simulink model "MGmono_rtiFPGASeparationFile"  (R2018b)
settings: Solver=FixedStepAuto  StartTime=0.0  StopTime=Inf  FixedStep=N*T  RelTol=1e-3
PostLoadFcn:
  | , if any(exist('dsrtsu_mdlpostloadfcn', 'file') ~= 0), dsrtsu_mdlpostloadfcn('Execute', bdroot); end,
InitFcn:
  | , if any(exist('dsmpb_private', 'file') ~= 0), dsmpb_private('dsmpb_mdlclblib', 'Init', bdroot); end,
values from neighbouring files (symbols this model uses):
  amp = 1    [param.m]
  fixedgain_i = 10*1000/(3*100)    (= 33.3333333333)    [param.m]
  fixedgain_vc1 = 10*10000/(3*100*2.5)    (= 133.333333333)    [param.m]
  fixedgain_vc2 = 10*10000/(3*100*2.5)    (= 133.333333333)    [param.m]
  fixedgain_vc3 = 10*22000/(3*100*2.5)    (= 293.333333333)    [param.m]
  fixedgain_vc4 = 10*22000/(3*100*2.5)    (= 293.333333333)    [param.m]
  fixedgain_vc5 = 10*22000/(3*100*2.5)    (= 293.333333333)    [param.m]
  freq = 50    [param.m]
  gain_iL1 = 1    [param.m]
  gain_iL2 = 1    [param.m]
  gain_iL3 = 1    [param.m]
  gain_iL4 = 1    [param.m]
  gain_vc1 = 1    [param.m]
  gain_vc2 = 1    [param.m]
  gain_vc3 = 1    [param.m]
  gain_vc4 = 1    [param.m]
  gain_vc5 = 1    [param.m]
  Ii = 10    [param.m]
  Ipv = 0.01    [param.m]
  Iv = 0.1    [param.m]
  Ki = 1e-7    (= 1e-07)    [param.m]
  Kp = 0.5    [param.m]
  maxd = N-1    (= 9)    [param.m]
  mind = 1    [param.m]
  N = 10    [param.m]
  offset_iL1 = 0.2    [param.m]
  offset_iL2 = 0.2    [param.m]
  offset_iL3 = -2e-3    (= -0.002)    [param.m]
  offset_iL4 = -2e-3    (= -0.002)    [param.m]
  offset_vc1 = -0.21    [param.m]
  offset_vc2 = -0.17    [param.m]
  offset_vc3 = 0.2    [param.m]
  offset_vc4 = -0.05    [param.m]
  offset_vc5 = -0.01    [param.m]
  Pi = 0.3    [param.m]
  Ppv = 0.05    [param.m]
  Pv = 0.01    [param.m]
  T = 6e-6    (= 6e-06)    [param.m]
  Tf = 1/1000    (= 0.001)    [param.m]
  Tfdc = 1/20    (= 0.05)    [param.m]
  v_dc_ref = 80    [param.m]
undefined symbols (not defined in the file or in its folder): DiscIntNeverNeededParam
libraries: xbsIndex_r4 x155, rti1202lib_adc_class1 x9, rtiproclib x7, simulink x6, rtifpgainterfacelib x1
(part 3 of 5)

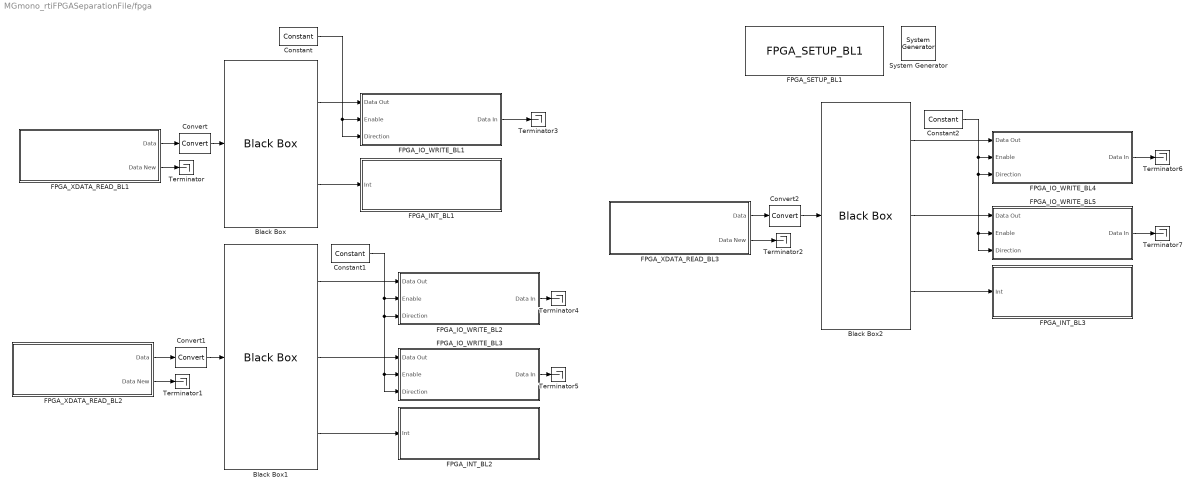
== system MGmono_rtiFPGASeparationFile/fpga ==
  " System Generator" : xbsIndex_r4/ System Generator  Tag=genX  xilinxfamily=kintex7  part=xc7k325t  speed=-3  package=fbg676  synthesis_tool=Vivado  clock_wrapper=Clock Enables  directory=./netlist  proj_type=Vivado  Synth_file=Vivado Synthesis Defaults  Impl_file=Vivado Implementation Defaults  testbench=off  simulink_period=1e-08  sysclk_period=10  dcm_input_clock_period=10  incr_netlist=off  trim_vbits=Everywhere in SubSystem  dbl_ovrd=According to Block Masks  core_generation=According to Block Masks  run_coregen=off  deprecated_control=off  eval_field=0  block_type=sysgen
  Black Box : xbsIndex_r4/Black Box  init_code=boost_config  sim_method=ISE Simulator  verbose=off  block_type=blackbox2
  Black Box1 : xbsIndex_r4/Black Box  init_code=halfbridge_config  sim_method=ISE Simulator  verbose=off  block_type=blackbox2
  Black Box2 : xbsIndex_r4/Black Box  init_code=hb_inv_config  sim_method=ISE Simulator  verbose=off  block_type=blackbox2
  Constant : xbsIndex_r4/Constant  const=1.0  gui_display_data_type=Fixed-point  arith_type=Signed (2's comp)  n_bits=16  bin_pt=14  preci_type=Single  exp_width=8  frac_width=24  explicit_period=off  period=1  equ=P=C  opselect=C  inp2=PCIN>>17  opr=+  inp1=P  carry=CIN  dbl_ovrd=off  block_type=constant
  Constant1 : xbsIndex_r4/Constant  const=1.0  gui_display_data_type=Fixed-point  arith_type=Signed (2's comp)  n_bits=16  bin_pt=14  preci_type=Single  exp_width=8  frac_width=24  explicit_period=off  period=1  equ=P=C  opselect=C  inp2=PCIN>>17  opr=+  inp1=P  carry=CIN  dbl_ovrd=off  block_type=constant
  Constant2 : xbsIndex_r4/Constant  const=1.0  gui_display_data_type=Fixed-point  arith_type=Signed (2's comp)  n_bits=16  bin_pt=14  preci_type=Single  exp_width=8  frac_width=24  explicit_period=off  period=1  equ=P=C  opselect=C  inp2=PCIN>>17  opr=+  inp1=P  carry=CIN  dbl_ovrd=off  block_type=constant
  Convert : xbsIndex_r4/Convert  gui_display_data_type=Fixed-point  arith_type=Unsigned  n_bits=10  bin_pt=0  float_type=Single  exp_bits=8  fraction_bits=24  quantization=Truncate  overflow=Wrap  en=off  latency=1  pipeline=off  dbl_ovrd=off  block_type=convert
  Convert1 : xbsIndex_r4/Convert  gui_display_data_type=Fixed-point  arith_type=Unsigned  n_bits=10  bin_pt=0  float_type=Single  exp_bits=8  fraction_bits=24  quantization=Truncate  overflow=Wrap  en=off  latency=1  pipeline=off  dbl_ovrd=off  block_type=convert
  Convert2 : xbsIndex_r4/Convert  gui_display_data_type=Fixed-point  arith_type=Unsigned  n_bits=10  bin_pt=0  float_type=Single  exp_bits=8  fraction_bits=24  quantization=Truncate  overflow=Wrap  en=off  latency=1  pipeline=off  dbl_ovrd=off  block_type=convert
  FPGA_INT_BL1 : Subsystem  LoadFcn=try, rti_fpga_blk_loadfcn(gcbh); catch,errordlg({lasterr, '','Please check your RTI installation.'},['Error: ' upper(bdroot)], 'replace'); end  InitFcn=try, rti_fpga_blk_initfcn(gcbh); catch,errordlg({lasterr, '','Please check your RTI installation.'},['Error: ' upper(bdroot)], 'replace'); end  StartFcn=try, rti_fpga_blk_startfcn(gcbh); catch,errordlg({lasterr, '','Please check your RTI installation.'},['Error: ' upper(bdroot)], 'replace'); end  mask(RTI){DSProperties=struct('RTI',struct('Version',uint32(4),'BlockType',struct('isSLSource',uint8(0),'isSLSink',uint8(0),'isHWSource',uint8(0),'isHWSink',uint8(0),'isSetup',uint8(1),'isInline',uint8(1),'isNonInline',uint8(0),'isInterrupt',uint8(0),'isChannelwise',uint8(0)),'IOBoardType','DSFPGA','UnitType','','Identifier','INT','DialogType','ML','BlockSet','FPGA','SlaveProcessor','')), RTIBlockInterface=struct('InputPortsActive',1,'InputPortsWidth',int32(1),'InputPortsDataType',{{'SS_DOUBLE'}},'InputPortsName',{{'Int'}},'InitLevel',3,'DialogFcn','rtifpgaintgui','BlockDisplay',{{'Interrupt','auto'}},'IconTransparency','on','BlockName',struct('Token',{{'FPGA_INT_BL1'}})), RTIBlockParameters=struct('BoardNo',{{1,'OFF',[1 16]}},'Name',{{['Interrupt 1'],'OFF',[]}},'CustomName',{{['int_pv '],'OFF',[]}},'AccessTyp',{{'Interrupt','OFF',[]}},'ChannelNo',{{'1','OFF',[]}},'FrmIni',{{'fpga_framework_ini_DS1302_XC7K325T_FLEXIBLEIO','OFF',[]}},'DynFcn',{{struct('GUIPar',struct('Name',{{['Enable simulation port']},{'Used'}},'GUIType',{{'checkbox'},{'none'}},'Range',{{'0','1'},{'0','1'}},'Init',{{'0'},{'1','0'}},'Group',{{''},{''}},'Generic',{{''},{'usr_int_00_used'}},'Application',{{'ApplicationIn(1).Show'},{''}},'Framework',{{''},{''}},'Callback',{{''},{''}}),'Exl',{{''}},'HlpFile',{{'rtifpga','INT_OUT_DS1302'}},'Hlp',{{['Click below for further details on this I/O function.']}},'Gen',struct('name',{'','usr_int_00_used'},'value',{'','1'},'unusedinit',{'','0'},'tag',{'',''},'filename',{'',''}),'Frm',struct('FrameworkOut',struct('Name',{{'usr_interrupt_00'}},'BitWidth',{{'1'}},'BinaryPoint',{{'0'}},'Format',{{'unsigned'}}),'FrameworkIn',struct('Name',{},'BitWidth',{},'BinaryPoint',{},'Format',{})),'App',struct('ApplicationOut',struct('Name',{{'Int'}},'Show',{{true}}),'ApplicationIn',struct('Name',{{'Sim_Int'}},'Show',{{0}})),'Con',{{'FrameworkOut(1)','ApplicationOut(1)'}},'OffCon',{{'data_i','FrameworkOut(1)','data_o','ApplicationIn(1)'}},'OffModel',{{'phs_interrupt'}}),'OFF',[]}},'FPGAFrameworkId',{{'8','OFF',[]}},'CorrBlock',{{struct('Data','','DataTag',''),'OFF',[]}}), RTISFcnParameters=struct('BoardNo','double'), RTIBlockParaDefault=struct('BoardNo',1,'Name',[' '],'CustomName',[' '],'AccessTyp',['<not selected>'],'ChannelNo',['<not selected>'],'FrmIni',[' '],'DynFcn',struct('GUIPar','','Hlp','','HlpFile','','Frm','','Gen','','Exl','','App','','Con',''),'FPGAFrameworkId',[' '],'CorrBlock',struct('Data','','DataTag',''))}
      mask init:
      | % blkh = gcbh;
      | % [sfi, sfp, sfpt] = rti_fpga_blockinitial(blkh,'UPDATEPARAMETER');
      | % rti_fpga_blockinitial(blkh,'UPDATEBLOCKGUI');
      settings: CopyFcn=try, rti_fpga_blk_copyfcn(gcbh); catch,errordlg({lasterr, '','Please check your RTI installation.'},['Error: ' upper(bdroot)], 'replace'); end  DeleteFcn=try, rti_fpga_blk_deletefcn(gcbh); catch,errordlg({lasterr, '','Please check your RTI installation.'},['Error: ' upper(bdroot)], 'replace'); end  ModelCloseFcn=try, rti_fpga_blk_modelclosefcn(gcbh); catch,errordlg({lasterr, '','Please check your RTI installation.'},['Error: ' upper(bdroot)], 'replace'); end  PreSaveFcn=try, rti_fpga_blk_presavefcn(gcbh); catch,errordlg({lasterr, '','Please check your RTI installation.'},['Error: ' upper(bdroot)], 'replace'); end  NameChangeFcn=try, rti_fpga_blk_namechangefcn(gcbh); catch,errordlg({lasterr, '','Please check your RTI installation.'},['Error: ' upper(bdroot)], 'replace'); end  OpenFcn=try, rti_fpga_blk_openfcn(gcbh); catch,errordlg({lasterr, '','Please check your RTI installation.'},['Error: ' upper(bdroot)], 'replace'); end  CloseFcn=try, rti_fpga_blk_closefcn(gcbh); catch,errordlg({lasterr, '','Please check your RTI installation.'},['Error: ' upper(bdroot)], 'replace'); end  ParentCloseFcn=try, rti_fpga_blk_parentclosefcn(gcbh); catch,errordlg({lasterr, '','Please check your RTI installation.'},['Error: ' upper(bdroot)], 'replace'); end
      mask Help: eval( ['lasterror(''reset''); rtifpgaguilib(''RTIMaskHelp'', gcbh);', 'disp(lasterr);']);
      mask Display: text(0.5,0.575,'Interrupt 1','HorizontalAlignment','center');text(0.5,0.425,'int_pv ','HorizontalAlignment','center');
  FPGA_INT_BL2 : Subsystem  LoadFcn=try, rti_fpga_blk_loadfcn(gcbh); catch,errordlg({lasterr, '','Please check your RTI installation.'},['Error: ' upper(bdroot)], 'replace'); end  InitFcn=try, rti_fpga_blk_initfcn(gcbh); catch,errordlg({lasterr, '','Please check your RTI installation.'},['Error: ' upper(bdroot)], 'replace'); end  StartFcn=try, rti_fpga_blk_startfcn(gcbh); catch,errordlg({lasterr, '','Please check your RTI installation.'},['Error: ' upper(bdroot)], 'replace'); end  mask(RTI){DSProperties=struct('RTI',struct('Version',uint32(4),'BlockType',struct('isSLSource',uint8(0),'isSLSink',uint8(0),'isHWSource',uint8(0),'isHWSink',uint8(0),'isSetup',uint8(1),'isInline',uint8(1),'isNonInline',uint8(0),'isInterrupt',uint8(0),'isChannelwise',uint8(0)),'IOBoardType','DSFPGA','UnitType','','Identifier','INT','DialogType','ML','BlockSet','FPGA','SlaveProcessor','')), RTIBlockInterface=struct('InputPortsActive',1,'InputPortsWidth',int32(1),'InputPortsDataType',{{'SS_DOUBLE'}},'InputPortsName',{{'Int'}},'InitLevel',3,'DialogFcn','rtifpgaintgui','BlockDisplay',{{'Interrupt','auto'}},'IconTransparency','on','BlockName',struct('Token',{{'FPGA_INT_BL1'}})), RTIBlockParameters=struct('BoardNo',{{1,'OFF',[1 16]}},'Name',{{['Interrupt 2'],'OFF',[]}},'CustomName',{{'int_bat','OFF',[]}},'AccessTyp',{{'Interrupt','OFF',[]}},'ChannelNo',{{'2','OFF',[]}},'FrmIni',{{'fpga_framework_ini_DS1302_XC7K325T_FLEXIBLEIO','OFF',[]}},'DynFcn',{{struct('GUIPar',struct('Name',{{['Enable simulation port']},{'Used'}},'GUIType',{{'checkbox'},{'none'}},'Range',{{'0','1'},{'0','1'}},'Init',{{'0'},{'1','0'}},'Group',{{''},{''}},'Generic',{{''},{'usr_int_01_used'}},'Application',{{'ApplicationIn(1).Show'},{''}},'Framework',{{''},{''}},'Callback',{{''},{''}}),'Exl',{{''}},'HlpFile',{{'rtifpga','INT_OUT_DS1302'}},'Hlp',{{['Click below for further details on this I/O function.']}},'Gen',struct('name',{'','usr_int_01_used'},'value',{'','1'},'unusedinit',{'','0'},'tag',{'',''},'filename',{'',''}),'Frm',struct('FrameworkOut',struct('Name',{{'usr_interrupt_01'}},'BitWidth',{{'1'}},'BinaryPoint',{{'0'}},'Format',{{'unsigned'}}),'FrameworkIn',struct('Name',{},'BitWidth',{},'BinaryPoint',{},'Format',{})),'App',struct('ApplicationOut',struct('Name',{{'Int'}},'Show',{{true}}),'ApplicationIn',struct('Name',{{'Sim_Int'}},'Show',{{0}})),'Con',{{'FrameworkOut(1)','ApplicationOut(1)'}},'OffCon',{{'data_i','FrameworkOut(1)','data_o','ApplicationIn(1)'}},'OffModel',{{'phs_interrupt'}}),'OFF',[]}},'FPGAFrameworkId',{{'8','OFF',[]}},'CorrBlock',{{struct('Data','','DataTag',''),'OFF',[]}}), RTISFcnParameters=struct('BoardNo','double'), RTIBlockParaDefault=struct('BoardNo',1,'Name',[' '],'CustomName',[' '],'AccessTyp',['<not selected>'],'ChannelNo',['<not selected>'],'FrmIni',[' '],'DynFcn',struct('GUIPar','','Hlp','','HlpFile','','Frm','','Gen','','Exl','','App','','Con',''),'FPGAFrameworkId',[' '],'CorrBlock',struct('Data','','DataTag',''))}
      mask init:
      | % blkh = gcbh;
      | % [sfi, sfp, sfpt] = rti_fpga_blockinitial(blkh,'UPDATEPARAMETER');
      | % rti_fpga_blockinitial(blkh,'UPDATEBLOCKGUI');
      settings: CopyFcn=try, rti_fpga_blk_copyfcn(gcbh); catch,errordlg({lasterr, '','Please check your RTI installation.'},['Error: ' upper(bdroot)], 'replace'); end  DeleteFcn=try, rti_fpga_blk_deletefcn(gcbh); catch,errordlg({lasterr, '','Please check your RTI installation.'},['Error: ' upper(bdroot)], 'replace'); end  ModelCloseFcn=try, rti_fpga_blk_modelclosefcn(gcbh); catch,errordlg({lasterr, '','Please check your RTI installation.'},['Error: ' upper(bdroot)], 'replace'); end  PreSaveFcn=try, rti_fpga_blk_presavefcn(gcbh); catch,errordlg({lasterr, '','Please check your RTI installation.'},['Error: ' upper(bdroot)], 'replace'); end  NameChangeFcn=try, rti_fpga_blk_namechangefcn(gcbh); catch,errordlg({lasterr, '','Please check your RTI installation.'},['Error: ' upper(bdroot)], 'replace'); end  OpenFcn=try, rti_fpga_blk_openfcn(gcbh); catch,errordlg({lasterr, '','Please check your RTI installation.'},['Error: ' upper(bdroot)], 'replace'); end  CloseFcn=try, rti_fpga_blk_closefcn(gcbh); catch,errordlg({lasterr, '','Please check your RTI installation.'},['Error: ' upper(bdroot)], 'replace'); end  ParentCloseFcn=try, rti_fpga_blk_parentclosefcn(gcbh); catch,errordlg({lasterr, '','Please check your RTI installation.'},['Error: ' upper(bdroot)], 'replace'); end
      mask Help: eval( ['lasterror(''reset''); rtifpgaguilib(''RTIMaskHelp'', gcbh);', 'disp(lasterr);']);
      mask Display: text(0.5,0.575,'Interrupt 2','HorizontalAlignment','center');text(0.5,0.425,'int_bat','HorizontalAlignment','center');
  FPGA_INT_BL3 : Subsystem  LoadFcn=try, rti_fpga_blk_loadfcn(gcbh); catch,errordlg({lasterr, '','Please check your RTI installation.'},['Error: ' upper(bdroot)], 'replace'); end  InitFcn=try, rti_fpga_blk_initfcn(gcbh); catch,errordlg({lasterr, '','Please check your RTI installation.'},['Error: ' upper(bdroot)], 'replace'); end  StartFcn=try, rti_fpga_blk_startfcn(gcbh); catch,errordlg({lasterr, '','Please check your RTI installation.'},['Error: ' upper(bdroot)], 'replace'); end  mask(RTI){DSProperties=struct('RTI',struct('Version',uint32(4),'BlockType',struct('isSLSource',uint8(0),'isSLSink',uint8(0),'isHWSource',uint8(0),'isHWSink',uint8(0),'isSetup',uint8(1),'isInline',uint8(1),'isNonInline',uint8(0),'isInterrupt',uint8(0),'isChannelwise',uint8(0)),'IOBoardType','DSFPGA','UnitType','','Identifier','INT','DialogType','ML','BlockSet','FPGA','SlaveProcessor','')), RTIBlockInterface=struct('InputPortsActive',1,'InputPortsWidth',int32(1),'InputPortsDataType',{{'SS_DOUBLE'}},'InputPortsName',{{'Int'}},'InitLevel',3,'DialogFcn','rtifpgaintgui','BlockDisplay',{{'Interrupt','auto'}},'IconTransparency','on','BlockName',struct('Token',{{'FPGA_INT_BL1'}})), RTIBlockParameters=struct('BoardNo',{{1,'OFF',[1 16]}},'Name',{{['Interrupt 3'],'OFF',[]}},'CustomName',{{'int_inv','OFF',[]}},'AccessTyp',{{'Interrupt','OFF',[]}},'ChannelNo',{{'3','OFF',[]}},'FrmIni',{{'fpga_framework_ini_DS1302_XC7K325T_FLEXIBLEIO','OFF',[]}},'DynFcn',{{struct('GUIPar',struct('Name',{{['Enable simulation port']},{'Used'}},'GUIType',{{'checkbox'},{'none'}},'Range',{{'0','1'},{'0','1'}},'Init',{{'0'},{'1','0'}},'Group',{{''},{''}},'Generic',{{''},{'usr_int_02_used'}},'Application',{{'ApplicationIn(1).Show'},{''}},'Framework',{{''},{''}},'Callback',{{''},{''}}),'Exl',{{''}},'HlpFile',{{'rtifpga','INT_OUT_DS1302'}},'Hlp',{{['Click below for further details on this I/O function.']}},'Gen',struct('name',{'','usr_int_02_used'},'value',{'','1'},'unusedinit',{'','0'},'tag',{'',''},'filename',{'',''}),'Frm',struct('FrameworkOut',struct('Name',{{'usr_interrupt_02'}},'BitWidth',{{'1'}},'BinaryPoint',{{'0'}},'Format',{{'unsigned'}}),'FrameworkIn',struct('Name',{},'BitWidth',{},'BinaryPoint',{},'Format',{})),'App',struct('ApplicationOut',struct('Name',{{'Int'}},'Show',{{true}}),'ApplicationIn',struct('Name',{{'Sim_Int'}},'Show',{{0}})),'Con',{{'FrameworkOut(1)','ApplicationOut(1)'}},'OffCon',{{'data_i','FrameworkOut(1)','data_o','ApplicationIn(1)'}},'OffModel',{{'phs_interrupt'}}),'OFF',[]}},'FPGAFrameworkId',{{'8','OFF',[]}},'CorrBlock',{{struct('Data','','DataTag',''),'OFF',[]}}), RTISFcnParameters=struct('BoardNo','double'), RTIBlockParaDefault=struct('BoardNo',1,'Name',[' '],'CustomName',[' '],'AccessTyp',['<not selected>'],'ChannelNo',['<not selected>'],'FrmIni',[' '],'DynFcn',struct('GUIPar','','Hlp','','HlpFile','','Frm','','Gen','','Exl','','App','','Con',''),'FPGAFrameworkId',[' '],'CorrBlock',struct('Data','','DataTag',''))}
      mask init:
      | % blkh = gcbh;
      | % [sfi, sfp, sfpt] = rti_fpga_blockinitial(blkh,'UPDATEPARAMETER');
      | % rti_fpga_blockinitial(blkh,'UPDATEBLOCKGUI');
      settings: CopyFcn=try, rti_fpga_blk_copyfcn(gcbh); catch,errordlg({lasterr, '','Please check your RTI installation.'},['Error: ' upper(bdroot)], 'replace'); end  DeleteFcn=try, rti_fpga_blk_deletefcn(gcbh); catch,errordlg({lasterr, '','Please check your RTI installation.'},['Error: ' upper(bdroot)], 'replace'); end  ModelCloseFcn=try, rti_fpga_blk_modelclosefcn(gcbh); catch,errordlg({lasterr, '','Please check your RTI installation.'},['Error: ' upper(bdroot)], 'replace'); end  PreSaveFcn=try, rti_fpga_blk_presavefcn(gcbh); catch,errordlg({lasterr, '','Please check your RTI installation.'},['Error: ' upper(bdroot)], 'replace'); end  NameChangeFcn=try, rti_fpga_blk_namechangefcn(gcbh); catch,errordlg({lasterr, '','Please check your RTI installation.'},['Error: ' upper(bdroot)], 'replace'); end  OpenFcn=try, rti_fpga_blk_openfcn(gcbh); catch,errordlg({lasterr, '','Please check your RTI installation.'},['Error: ' upper(bdroot)], 'replace'); end  CloseFcn=try, rti_fpga_blk_closefcn(gcbh); catch,errordlg({lasterr, '','Please check your RTI installation.'},['Error: ' upper(bdroot)], 'replace'); end  ParentCloseFcn=try, rti_fpga_blk_parentclosefcn(gcbh); catch,errordlg({lasterr, '','Please check your RTI installation.'},['Error: ' upper(bdroot)], 'replace'); end
      mask Help: eval( ['lasterror(''reset''); rtifpgaguilib(''RTIMaskHelp'', gcbh);', 'disp(lasterr);']);
      mask Display: text(0.5,0.575,'Interrupt 3','HorizontalAlignment','center');text(0.5,0.425,'int_inv','HorizontalAlignment','center');
  FPGA_IO_WRITE_BL1 : Subsystem  LoadFcn=try, rti_fpga_blk_loadfcn(gcbh); catch,errordlg({lasterr, '','Please check your RTI installation.'},['Error: ' upper(bdroot)], 'replace'); end  InitFcn=try, rti_fpga_blk_initfcn(gcbh); catch,errordlg({lasterr, '','Please check your RTI installation.'},['Error: ' upper(bdroot)], 'replace'); end  StartFcn=try, rti_fpga_blk_startfcn(gcbh); catch,errordlg({lasterr, '','Please check your RTI installation.'},['Error: ' upper(bdroot)], 'replace'); end  mask(RTI){DSProperties=struct('RTI',struct('Version',uint32(6),'BlockType',struct('isSLSource',uint8(0),'isSLSink',uint8(0),'isHWSource',uint8(0),'isHWSink',uint8(0),'isSetup',uint8(1),'isInline',uint8(1),'isNonInline',uint8(0),'isInterrupt',uint8(0),'isChannelwise',uint8(0)),'IOBoardType','DSFPGA','UnitType','','Identifier','IOWRITE','DialogType','ML','BlockSet','FPGA','SlaveProcessor','')), RTIBlockInterface=struct('InputPortsActive',1,'InputPortsWidth',int32(1),'InputPortsDataType',{{'SS_DOUBLE'}},'InputPortsName',{{['To IO']}},'InitLevel',3,'DialogFcn','rtifpgaiowritegui','BlockDisplay',{{['FPGA IO Write'],'auto'}},'IconTransparency','on','BlockName',struct('Token',{{'FPGA_IO_Write_BL1'}})), RTIBlockParameters=struct('BoardNo',{{1,'OFF',[1 16]}},'IOType',{{'All','OFF',[]}},'ChannelNo',{{'2','OFF',[]}},'FrmIni',{{'fpga_framework_ini_DS1302_XC7K325T_FLEXIBLEIO','OFF',[]}},'IOFrmIni',{{'','OFF',[]}},'Name',{{['Digital InOut 2 (Class 1)'],'OFF',[]}},'DynFcn',{{struct('GUIPar',struct('Name',{{'Used'},{['Invert values']},{['Input filter (0ns..10,000,000ns)']},{['Input filter calculated']},{['High supply']},{['Rising edge delay (0ns..655350ns)']},{['Enable digital out simulation port']},{['Enable digital in simulation port']},{['Rising edge delay calculated']},{['Invert input polarity']},{['Invert output polarity']},{['Enable FPGA test access and scaling for this block']}},'GUIType',{{'none'},{'popup','Off','On'},{'edit'},{'none'},{'popup','5V','3.3V','2.5V'},{'edit'},{'checkbox'},{'checkbox'},{'none'},{'popup','Disabled','Enabled'},{'popup','Disabled','Enabled'},{'checkbox'}},'Range',{{'0','1'},{'0','1'},{''},{[0 1 2 3 4 5 6 7 8 9 10 11 12 13 14 15 16 17 18 19 20 21 22 23 24 25 26 27 28 29 30 31 32 33 34 35 36 37 38 39 40 41 42 43 44 45 46 47 48 49 50 51 52 53 54 55 56 57 58 59 60 61 62 63 64 65 66 67 68 69 70 71 72 73 74 75 76 77 78 79 80 81 82 83 84 85 86 87 88 89 90 91 92 93 94 95 96 97 98 99 100 101 102 103 104 105 106 107 108 109 110 111 112 113 114 115 116 117 118 119 120 121 122 123 124 125 126 127 128 129 130 131 132 133 134 135 136 137 138 139 140 141 142 143 144 145 146 147 148 149 150 151 152 153 154 155 156 157 158 159 160 161 162 163 164 165 166 167 168 169 170 171 172 173 174 175 176 177 178 179 180 181 182 183 184 185 186 187 188 189 190 191 192 193 194 195 196 197 198 199 200 201 202 203 204 205 206 207 208 209 210 211 212 213 214 215 216 217 218 219 220 221 222 223 224 225 226 227 228 229 230 231 232 233 234 235 236 237 238 239 240 241 242 243 244 245 246 247 248 249 250 251 252 253 254 255 256 257 258 259 260 261 262 263 264 265 266 267 268 269 270 271 272 273 274 275 276 277 278 279 280 281 282 283 284 285 286 287 288 289 290 291 292 293 294 295 296 297 298 299 300 301 302 303 304 305 306 307 308 309 310 311 312 313 314 315 316 317 318 319 320 321 322 323 324 325 326 327 328 329 330 331 332 333 334 335 336 337 338 339 340 341 342 343 344 345 346 347 348 349 350 351 352 353 354 355 356 357 358 359 360 361 362 363 364 365 366 367 368 369 370 371 372 373 374 375 376 377 378 379 380 381 382 383 384 385 386 387 388 389 390 391 392 393 394 395 396 397 398 399 400 401 402 403 404 405 406 407 408 409 410 411 412 413 414 415 416 417 418 419 420 421 422 423 424 425 426 427 428 429 430 431 432 433 434 435 436 437 438 439 440 441 442 443 444 445 446 447 448 449 450 451 452 453 454 455 456 457 458 459 460 461 462 463 464 465 466 467 468 469 470 471 472 473 474 475 476 477 478 479 480 481 482 483 484 485 486 487 488 489 490 491 492 493 494 495 496 497 498 499 500 501 502 503 504 505 506 507 508 509 510 511]},{'0','1','2'},{''},{'0','1'},{'0','1'},{[0 1 2 3 4 5 6 7 8 9 10 11 12 13 14 15 16 17 18 19 20 21 22 23 24 25 26 27 28 29 30 31 32 33 34 35 36 37 38 39 40 41 42 43 44 45 46 47 48 49 50 51 52 53 54 55 56 57 58 59 60 61 62 63 64 65 66 67 68 69 70 71 72 73 74 75 76 77 78 79 80 81 82 83 84 85 86 87 88 89 90 91 92 93 94 95 96 97 98 99 100 101 102 103 104 105 106 107 108 109 110 111 112 113 114 115 116 117 118 119 120 121 122 123 124 125 126 127 128 129 130 131 132 133 134 135 136 137 138 139 140 141 142 143 144 145 146 147 148 149 150 151 152 153 154 155 156 157 158 159 160 161 162 163 164 165 166 167 168 169 170 171 172 173 174 175 176 177 178 179 180 181 182 183 184 185 186 187 188 189 190 191 192 193 194 195 196 197 198 199 200 201 202 203 204 205 206 207 208 209 210 211 212 213 214 215 216 217 218 219 220 221 222 223 224 225 226 227 228 229 230 231 232 233 234 235 236 237 238 239 240 241 242 243 244 245 246 247 248 249 250 251 252 253 254 255 256 257 258 259 260 261 262 263 264 265 266 267 268 269 270 271 272 273 274 275 276 277 278 279 280 281 282 283 284 285 286 287 288 289 290 291 292 293 294 295 296 297 298 299 300 301 302 303 304 305 306 307 308 309 310 311 312 313 314 315 316 317 318 319 320 321 322 323 324 325 326 327 328 329 330 331 332 333 334 335 336 337 338 339 340 341 342 343 344 345 346 347 348 349 350 351 352 353 354 355 356 357 358 359 360 361 362 363 364 365 366 367 368 369 370 371 372 373 374 375 376 377 378 379 380 381 382 383 384 385 386 387 388 389 390 391 392 393 394 395 396 397 398 399 400 401 402 403 404 405 406 407 408 409 410 411 412 413 414 415 416 417 418 419 420 421 422 423 424 425 426 427 428 429 430 431 432 433 434 435 436 437 438 439 440 441 442 443 444 445 446 447 448 449 450 451 452 453 454 455 456 457 458 459 460 461 462 463 464 465 466 467 468 469 470 471 472 473 474 475 476 477 478 479 480 481 482 483 484 485 486 487 488 489 490 491 492 493 494 495 496 497 498 499 500 501 502 503 504 505 506 507 508 509 510 511 512 513 514 515 516 517 518 519 520 521 522 523 524 525 526 527 528 529 530 531 532 533 534 535 536 537 538 539 540 541 542 543 544 545 546 547 548 549 550 551 552 553 554 555 556 557 558 559 560 561 562 563 564 565 566 567 568 569 570 571 572 573 574 575 576 577 578 579 580 581 582 583 584 585 586 587 588 589 590 591 592 593 594 595 596 597 598 599 600 601 602 603 604 605 606 607 608 609 610 611 612 613 614 615 616 617 618 619 620 621 622 623 624 625 626 627 628 629 630 631 632 633 634 635 636 637 638 639 640 641 642 643 644 645 646 647 648 649 650 651 652 653 654 655 656 657 658 659 660 661 662 663 664 665 666 667 668 669 670 671 672 673 674 675 676 677 678 679 680 681 682 683 684 685 686 687 688 689 690 691 692 693 694 695 696 697 698 699 700 701 702 703 704 705 706 707 708 709 710 711 712 713 714 715 716 717 718 719 720 721 722 723 724 725 726 727 728 729 730 731 732 733 734 735 736 737 738 739 740 741 742 743 744 745 746 747 748 749 750 751 752 753 754 755 756 757 758 759 760 761 762 763 764 765 766 767 768 769 770 771 772 773 774 775 776 777 778 779 780 781 782 783 784 785 786 787 788 789 790 791 792 793 794 795 796 797 798 799 800 801 802 803 804 805 806 807 808 809 810 811 812 813 814 815 816 817 818 819 820 821 822 823 824 825 826 827 828 829 830 831 832 833 834 835 836 837 838 839 840 841 842 843 844 845 846 847 848 849 850 851 852 853 854 855 856 857 858 859 860 861 862 863 864 865 866 867 868 869 870 871 872 873 874 875 876 877 878 879 880 881 882 883 884 885 886 887 888 889 890 891 892 893 894 895 896 897 898 899 900 901 902 903 904 905 906 907 908 909 910 911 912 913 914 915 916 917 918 919 920 921 922 923 924 925 926 927 928 929 930 931 932 933 934 935 936 937 938 939 940 941 942 943 944 945 946 947 948 949 950 951 952 953 954 955 956 957 958 959 960 961 962 963 964 965 966 967 968 969 970 971 972 973 974 975 976 977 978 979 980 981 982 983 984 985 986 987 988 989 990 991 992 993 994 995 996 997 998 999 1000 1001 1002 1003 1004 1005 1006 1007 1008 1009 1010 1011 1012 1013 1014 1015 1016 1017 1018 1019 1020 ...(+378111 chars)]},{'0','1'},{'0','1'},{'0','1'}},'Init',{{'1','0'},{'0'},{'0'},{'0'},{'0'},{'0'},{'0'},{'0'},{'0'},{'0'},{'0'},{'1'}},'Group',{{''},{''},{''},{''},{''},{''},{''},{''},{''},{''},{''},{''}},'Generic',{{'diotp1_01_used'},{'diotp1_01_invert'},{'DIGINOUT_01FILTER'},{'diotp1_01_filter'},{'diotp1_01_voltage'},{'DIGINOUT_01_DELAY'},{''},{''},{'diotp1_01_delay'},{'RTIFPGA_INVERT_INPUT_POLARITY(01)'},{'RTIFPGA_INVERT_OUTPUT_POLARITY(01)'},{'RTIFPGA_TA_SCALING_ENABLE(01)'}},'Application',{{''},{''},{''},{''},{''},{''},{'ApplicationIn(2).Show'},{'ApplicationOut(4).Show'},{''},{''},{''},{''}},'Framework',{{''},{''},{''},{''},{''},{''},{''},{''},{''},{''},{''},{''}},'Callback',{{''},{''},{'fpga_framework_ini_DS1302_XC7K325T_FLEXIBLEIO:input_filter_calculation'},{''},{''},{'fpga_framework_ini_DS1302_XC7K325T_FLEXIBLEIO:rising_edge_delay_calculation'},{''},{''},{''},{''},{''},{''}},'Tab',{[],[],[],[],[],[],[],[],[],{'3'},{'3'},{'3'}},'Tag',{[],[],[],[],[],[],[],[],[],[],[],{''}},'Value',{{'1'},{'0'},{'0'},{'0'},{'0'},{'0'},{0},{0},{'0'},{'0'},{'0'},{'1'}}),'Exl',{{''}},'HlpFile',{{'rtifpga','DIGITAL_INOUT_CL1_DS1302'}},'Hlp',{{['Click below for further details on this I/O function.']}},'Gen',struct('name',{'diotp1_01_used','diotp1_01_invert','DIGINOUT_01FILTER','diotp1_01_filter','diotp1_01_voltage','DIGINOUT_01_DELAY','','','diotp1_01_delay','RTIFPGA_INVERT_INPUT_POLARITY(01)','RTIFPGA_INVERT_OUTPUT_POLARITY(01)','RTIFPGA_TA_SCALING_ENABLE(01)'},'value',{'1','0','0','0','0','0','','','0','0','0','1'},'unusedinit',{'0','','','','','','','','','','',''},'tag',{'','','','','','','','','','','',''},'filename',{'','','','','','','','','','','',''}),'Frm',struct('FrameworkOut',struct('Name',{{'diotp1_01_out'},{'diotp1_01_ena'},{'diotp1_01_dir'}},'BitWidth',{{'1'},{'1'},{'1'}},'BinaryPoint',{{'0'},{'0'},{'0'}},'Format',{{'unsigned'},{'unsigned'},{'unsigned'}},'Invert',{{'0'},[],[]},'RplcV',{{'0'},{'0'},{'0'}},'SwchV',{{'0'},{'0'},{'0'}}),'FrameworkIn',struct('Name',{{'diotp1_01_in'}},'BitWidth',{{'1'}},'BinaryPoint',{{'0'}},'Format',{{'unsigned'}},'Invert',{{'0'}},'RplcV',{{'0'}},'SwchV',{{'0'}})),'App',struct('ApplicationOut',struct('Name',{{['Data Out']},{'Enable'},{'Direction'},{['Sim Data In']}},'Show',{{true},{true},{true},{0}}),'ApplicationIn',struct('Name',{{['Data In']},{['Sim Data Out']}},'Show',{{true},{0}})),'Con',{{'FrameworkIn(1)','ApplicationIn(1)','FrameworkOut(1)','ApplicationOut(1)','FrameworkOut(2)','ApplicationOut(2)','FrameworkOut(3)','ApplicationOut(3)'}},'OffCon',{{'data_in_o','FrameworkIn(1)','data_in_i','ApplicationOut(4)','data_out_i','FrameworkOut(1)','data_out_o','ApplicationIn(2)','enable_i','FrameworkOut(2)','direction_i','FrameworkOut(3)'}},'OffModel',{{'dig_inout_tp1'}}),'OFF',[]}},'FPGAFrameworkId',{{'8','OFF',[]}},'CustomName',{{['s1 '],'OFF',[]}},'MGTFrmIni',{{'','OFF',[]}},'BusSettings',{{[' '],'OFF',[]}}), RTISFcnParameters=struct('BoardNo','double'), RTIBlockParaDefault=struct('BoardNo',1,'IOType','All','ChannelNo',[' '],'FrmIni',[' '],'IOFrmIni',[' '],'Name',[' '],'DynFcn',struct('GUIPar','','Hlp','','HlpFile','','Exl','','Frm','','Gen','','App','','Con',''),'FPGAFrameworkId',[' '],'CustomName',[' '],'MGTFrmIni',[' '],'BusSettings',[' '])}
      mask init:
      | % blkh = gcbh;
      | % [sfi, sfp, sfpt] = rti_fpga_blockinitial(blkh,'UPDATEPARAMETER');
      | % rti_fpga_blockinitial(blkh,'UPDATEBLOCKGUI');
      settings: CopyFcn=try, rti_fpga_blk_copyfcn(gcbh); catch,errordlg({lasterr, '','Please check your RTI installation.'},['Error: ' upper(bdroot)], 'replace'); end  DeleteFcn=try, rti_fpga_blk_deletefcn(gcbh); catch,errordlg({lasterr, '','Please check your RTI installation.'},['Error: ' upper(bdroot)], 'replace'); end  ModelCloseFcn=try, rti_fpga_blk_modelclosefcn(gcbh); catch,errordlg({lasterr, '','Please check your RTI installation.'},['Error: ' upper(bdroot)], 'replace'); end  PreSaveFcn=try, rti_fpga_blk_presavefcn(gcbh); catch,errordlg({lasterr, '','Please check your RTI installation.'},['Error: ' upper(bdroot)], 'replace'); end  NameChangeFcn=try, rti_fpga_blk_namechangefcn(gcbh); catch,errordlg({lasterr, '','Please check your RTI installation.'},['Error: ' upper(bdroot)], 'replace'); end  OpenFcn=try, rti_fpga_blk_openfcn(gcbh); catch,errordlg({lasterr, '','Please check your RTI installation.'},['Error: ' upper(bdroot)], 'replace'); end  CloseFcn=try, rti_fpga_blk_closefcn(gcbh); catch,errordlg({lasterr, '','Please check your RTI installation.'},['Error: ' upper(bdroot)], 'replace'); end  ParentCloseFcn=try, rti_fpga_blk_parentclosefcn(gcbh); catch,errordlg({lasterr, '','Please check your RTI installation.'},['Error: ' upper(bdroot)], 'replace'); end
      mask Help: eval( ['lasterror(''reset''); rtifpgaguilib(''RTIMaskHelp'', gcbh);', 'disp(lasterr);']);
      mask Display: text(0.5,0.575,'Digital InOut 2 (Class 1)','HorizontalAlignment','center');text(0.5,0.425,'s1 ','HorizontalAlignment','center');
  FPGA_IO_WRITE_BL2 : Subsystem  LoadFcn=try, rti_fpga_blk_loadfcn(gcbh); catch,errordlg({lasterr, '','Please check your RTI installation.'},['Error: ' upper(bdroot)], 'replace'); end  InitFcn=try, rti_fpga_blk_initfcn(gcbh); catch,errordlg({lasterr, '','Please check your RTI installation.'},['Error: ' upper(bdroot)], 'replace'); end  StartFcn=try, rti_fpga_blk_startfcn(gcbh); catch,errordlg({lasterr, '','Please check your RTI installation.'},['Error: ' upper(bdroot)], 'replace'); end  mask(RTI){DSProperties=struct('RTI',struct('Version',uint32(6),'BlockType',struct('isSLSource',uint8(0),'isSLSink',uint8(0),'isHWSource',uint8(0),'isHWSink',uint8(0),'isSetup',uint8(1),'isInline',uint8(1),'isNonInline',uint8(0),'isInterrupt',uint8(0),'isChannelwise',uint8(0)),'IOBoardType','DSFPGA','UnitType','','Identifier','IOWRITE','DialogType','ML','BlockSet','FPGA','SlaveProcessor','')), RTIBlockInterface=struct('InputPortsActive',1,'InputPortsWidth',int32(1),'InputPortsDataType',{{'SS_DOUBLE'}},'InputPortsName',{{['To IO']}},'InitLevel',3,'DialogFcn','rtifpgaiowritegui','BlockDisplay',{{['FPGA IO Write'],'auto'}},'IconTransparency','on','BlockName',struct('Token',{{'FPGA_IO_Write_BL1'}})), RTIBlockParameters=struct('BoardNo',{{1,'OFF',[1 16]}},'IOType',{{'All','OFF',[]}},'ChannelNo',{{'3','OFF',[]}},'FrmIni',{{'fpga_framework_ini_DS1302_XC7K325T_FLEXIBLEIO','OFF',[]}},'IOFrmIni',{{'','OFF',[]}},'Name',{{['Digital InOut 3 (Class 1)'],'OFF',[]}},'DynFcn',{{struct('GUIPar',struct('Name',{{'Used'},{['Invert values']},{['Input filter (0ns..10,000,000ns)']},{['Input filter calculated']},{['High supply']},{['Rising edge delay (0ns..655350ns)']},{['Enable digital out simulation port']},{['Enable digital in simulation port']},{['Rising edge delay calculated']},{['Invert input polarity']},{['Invert output polarity']},{['Enable FPGA test access and scaling for this block']}},'GUIType',{{'none'},{'popup','Off','On'},{'edit'},{'none'},{'popup','5V','3.3V','2.5V'},{'edit'},{'checkbox'},{'checkbox'},{'none'},{'popup','Disabled','Enabled'},{'popup','Disabled','Enabled'},{'checkbox'}},'Range',{{'0','1'},{'0','1'},{''},{[0 1 2 3 4 5 6 7 8 9 10 11 12 13 14 15 16 17 18 19 20 21 22 23 24 25 26 27 28 29 30 31 32 33 34 35 36 37 38 39 40 41 42 43 44 45 46 47 48 49 50 51 52 53 54 55 56 57 58 59 60 61 62 63 64 65 66 67 68 69 70 71 72 73 74 75 76 77 78 79 80 81 82 83 84 85 86 87 88 89 90 91 92 93 94 95 96 97 98 99 100 101 102 103 104 105 106 107 108 109 110 111 112 113 114 115 116 117 118 119 120 121 122 123 124 125 126 127 128 129 130 131 132 133 134 135 136 137 138 139 140 141 142 143 144 145 146 147 148 149 150 151 152 153 154 155 156 157 158 159 160 161 162 163 164 165 166 167 168 169 170 171 172 173 174 175 176 177 178 179 180 181 182 183 184 185 186 187 188 189 190 191 192 193 194 195 196 197 198 199 200 201 202 203 204 205 206 207 208 209 210 211 212 213 214 215 216 217 218 219 220 221 222 223 224 225 226 227 228 229 230 231 232 233 234 235 236 237 238 239 240 241 242 243 244 245 246 247 248 249 250 251 252 253 254 255 256 257 258 259 260 261 262 263 264 265 266 267 268 269 270 271 272 273 274 275 276 277 278 279 280 281 282 283 284 285 286 287 288 289 290 291 292 293 294 295 296 297 298 299 300 301 302 303 304 305 306 307 308 309 310 311 312 313 314 315 316 317 318 319 320 321 322 323 324 325 326 327 328 329 330 331 332 333 334 335 336 337 338 339 340 341 342 343 344 345 346 347 348 349 350 351 352 353 354 355 356 357 358 359 360 361 362 363 364 365 366 367 368 369 370 371 372 373 374 375 376 377 378 379 380 381 382 383 384 385 386 387 388 389 390 391 392 393 394 395 396 397 398 399 400 401 402 403 404 405 406 407 408 409 410 411 412 413 414 415 416 417 418 419 420 421 422 423 424 425 426 427 428 429 430 431 432 433 434 435 436 437 438 439 440 441 442 443 444 445 446 447 448 449 450 451 452 453 454 455 456 457 458 459 460 461 462 463 464 465 466 467 468 469 470 471 472 473 474 475 476 477 478 479 480 481 482 483 484 485 486 487 488 489 490 491 492 493 494 495 496 497 498 499 500 501 502 503 504 505 506 507 508 509 510 511]},{'0','1','2'},{''},{'0','1'},{'0','1'},{[0 1 2 3 4 5 6 7 8 9 10 11 12 13 14 15 16 17 18 19 20 21 22 23 24 25 26 27 28 29 30 31 32 33 34 35 36 37 38 39 40 41 42 43 44 45 46 47 48 49 50 51 52 53 54 55 56 57 58 59 60 61 62 63 64 65 66 67 68 69 70 71 72 73 74 75 76 77 78 79 80 81 82 83 84 85 86 87 88 89 90 91 92 93 94 95 96 97 98 99 100 101 102 103 104 105 106 107 108 109 110 111 112 113 114 115 116 117 118 119 120 121 122 123 124 125 126 127 128 129 130 131 132 133 134 135 136 137 138 139 140 141 142 143 144 145 146 147 148 149 150 151 152 153 154 155 156 157 158 159 160 161 162 163 164 165 166 167 168 169 170 171 172 173 174 175 176 177 178 179 180 181 182 183 184 185 186 187 188 189 190 191 192 193 194 195 196 197 198 199 200 201 202 203 204 205 206 207 208 209 210 211 212 213 214 215 216 217 218 219 220 221 222 223 224 225 226 227 228 229 230 231 232 233 234 235 236 237 238 239 240 241 242 243 244 245 246 247 248 249 250 251 252 253 254 255 256 257 258 259 260 261 262 263 264 265 266 267 268 269 270 271 272 273 274 275 276 277 278 279 280 281 282 283 284 285 286 287 288 289 290 291 292 293 294 295 296 297 298 299 300 301 302 303 304 305 306 307 308 309 310 311 312 313 314 315 316 317 318 319 320 321 322 323 324 325 326 327 328 329 330 331 332 333 334 335 336 337 338 339 340 341 342 343 344 345 346 347 348 349 350 351 352 353 354 355 356 357 358 359 360 361 362 363 364 365 366 367 368 369 370 371 372 373 374 375 376 377 378 379 380 381 382 383 384 385 386 387 388 389 390 391 392 393 394 395 396 397 398 399 400 401 402 403 404 405 406 407 408 409 410 411 412 413 414 415 416 417 418 419 420 421 422 423 424 425 426 427 428 429 430 431 432 433 434 435 436 437 438 439 440 441 442 443 444 445 446 447 448 449 450 451 452 453 454 455 456 457 458 459 460 461 462 463 464 465 466 467 468 469 470 471 472 473 474 475 476 477 478 479 480 481 482 483 484 485 486 487 488 489 490 491 492 493 494 495 496 497 498 499 500 501 502 503 504 505 506 507 508 509 510 511 512 513 514 515 516 517 518 519 520 521 522 523 524 525 526 527 528 529 530 531 532 533 534 535 536 537 538 539 540 541 542 543 544 545 546 547 548 549 550 551 552 553 554 555 556 557 558 559 560 561 562 563 564 565 566 567 568 569 570 571 572 573 574 575 576 577 578 579 580 581 582 583 584 585 586 587 588 589 590 591 592 593 594 595 596 597 598 599 600 601 602 603 604 605 606 607 608 609 610 611 612 613 614 615 616 617 618 619 620 621 622 623 624 625 626 627 628 629 630 631 632 633 634 635 636 637 638 639 640 641 642 643 644 645 646 647 648 649 650 651 652 653 654 655 656 657 658 659 660 661 662 663 664 665 666 667 668 669 670 671 672 673 674 675 676 677 678 679 680 681 682 683 684 685 686 687 688 689 690 691 692 693 694 695 696 697 698 699 700 701 702 703 704 705 706 707 708 709 710 711 712 713 714 715 716 717 718 719 720 721 722 723 724 725 726 727 728 729 730 731 732 733 734 735 736 737 738 739 740 741 742 743 744 745 746 747 748 749 750 751 752 753 754 755 756 757 758 759 760 761 762 763 764 765 766 767 768 769 770 771 772 773 774 775 776 777 778 779 780 781 782 783 784 785 786 787 788 789 790 791 792 793 794 795 796 797 798 799 800 801 802 803 804 805 806 807 808 809 810 811 812 813 814 815 816 817 818 819 820 821 822 823 824 825 826 827 828 829 830 831 832 833 834 835 836 837 838 839 840 841 842 843 844 845 846 847 848 849 850 851 852 853 854 855 856 857 858 859 860 861 862 863 864 865 866 867 868 869 870 871 872 873 874 875 876 877 878 879 880 881 882 883 884 885 886 887 888 889 890 891 892 893 894 895 896 897 898 899 900 901 902 903 904 905 906 907 908 909 910 911 912 913 914 915 916 917 918 919 920 921 922 923 924 925 926 927 928 929 930 931 932 933 934 935 936 937 938 939 940 941 942 943 944 945 946 947 948 949 950 951 952 953 954 955 956 957 958 959 960 961 962 963 964 965 966 967 968 969 970 971 972 973 974 975 976 977 978 979 980 981 982 983 984 985 986 987 988 989 990 991 992 993 994 995 996 997 998 999 1000 1001 1002 1003 1004 1005 1006 1007 1008 1009 1010 1011 1012 1013 1014 1015 1016 1017 1018 1019 1020 ...(+378111 chars)]},{'0','1'},{'0','1'},{'0','1'}},'Init',{{'1','0'},{'0'},{'0'},{'0'},{'0'},{'0'},{'0'},{'0'},{'0'},{'0'},{'0'},{'1'}},'Group',{{''},{''},{''},{''},{''},{''},{''},{''},{''},{''},{''},{''}},'Generic',{{'diotp1_02_used'},{'diotp1_02_invert'},{'DIGINOUT_02FILTER'},{'diotp1_02_filter'},{'diotp1_02_voltage'},{'DIGINOUT_02_DELAY'},{''},{''},{'diotp1_02_delay'},{'RTIFPGA_INVERT_INPUT_POLARITY(02)'},{'RTIFPGA_INVERT_OUTPUT_POLARITY(02)'},{'RTIFPGA_TA_SCALING_ENABLE(02)'}},'Application',{{''},{''},{''},{''},{''},{''},{'ApplicationIn(2).Show'},{'ApplicationOut(4).Show'},{''},{''},{''},{''}},'Framework',{{''},{''},{''},{''},{''},{''},{''},{''},{''},{''},{''},{''}},'Callback',{{''},{''},{'fpga_framework_ini_DS1302_XC7K325T_FLEXIBLEIO:input_filter_calculation'},{''},{''},{'fpga_framework_ini_DS1302_XC7K325T_FLEXIBLEIO:rising_edge_delay_calculation'},{''},{''},{''},{''},{''},{''}},'Tab',{[],[],[],[],[],[],[],[],[],{'3'},{'3'},{'3'}},'Tag',{[],[],[],[],[],[],[],[],[],[],[],{''}}),'Exl',{{''}},'HlpFile',{{'rtifpga','DIGITAL_INOUT_CL1_DS1302'}},'Hlp',{{['Click below for further details on this I/O function.']}},'Gen',struct('name',{'diotp1_02_used','diotp1_02_invert','DIGINOUT_02FILTER','diotp1_02_filter','diotp1_02_voltage','DIGINOUT_02_DELAY','','','diotp1_02_delay','RTIFPGA_INVERT_INPUT_POLARITY(02)','RTIFPGA_INVERT_OUTPUT_POLARITY(02)','RTIFPGA_TA_SCALING_ENABLE(02)'},'value',{'1','0','0','0','0','0','','','0','0','0','1'},'unusedinit',{'0','','','','','','','','','','',''},'tag',{'','','','','','','','','','','',''},'filename',{'','','','','','','','','','','',''}),'Frm',struct('FrameworkOut',struct('Name',{{'diotp1_02_out'},{'diotp1_02_ena'},{'diotp1_02_dir'}},'BitWidth',{{'1'},{'1'},{'1'}},'BinaryPoint',{{'0'},{'0'},{'0'}},'Format',{{'unsigned'},{'unsigned'},{'unsigned'}},'Invert',{{'0'},[],[]},'RplcV',{{'0'},{'0'},{'0'}},'SwchV',{{'0'},{'0'},{'0'}}),'FrameworkIn',struct('Name',{{'diotp1_02_in'}},'BitWidth',{{'1'}},'BinaryPoint',{{'0'}},'Format',{{'unsigned'}},'Invert',{{'0'}},'RplcV',{{'0'}},'SwchV',{{'0'}})),'App',struct('ApplicationOut',struct('Name',{{['Data Out']},{'Enable'},{'Direction'},{['Sim Data In']}},'Show',{{true},{true},{true},{0}}),'ApplicationIn',struct('Name',{{['Data In']},{['Sim Data Out']}},'Show',{{true},{0}})),'Con',{{'FrameworkIn(1)','ApplicationIn(1)','FrameworkOut(1)','ApplicationOut(1)','FrameworkOut(2)','ApplicationOut(2)','FrameworkOut(3)','ApplicationOut(3)'}},'OffCon',{{'data_in_o','FrameworkIn(1)','data_in_i','ApplicationOut(4)','data_out_i','FrameworkOut(1)','data_out_o','ApplicationIn(2)','enable_i','FrameworkOut(2)','direction_i','FrameworkOut(3)'}},'OffModel',{{'dig_inout_tp1'}}),'OFF',[]}},'FPGAFrameworkId',{{'8','OFF',[]}},'CustomName',{{'s3','OFF',[]}},'MGTFrmIni',{{'','OFF',[]}},'BusSettings',{{[' '],'OFF',[]}}), RTISFcnParameters=struct('BoardNo','double'), RTIBlockParaDefault=struct('BoardNo',1,'IOType','All','ChannelNo',[' '],'FrmIni',[' '],'IOFrmIni',[' '],'Name',[' '],'DynFcn',struct('GUIPar','','Hlp','','HlpFile','','Exl','','Frm','','Gen','','App','','Con',''),'FPGAFrameworkId',[' '],'CustomName',[' '],'MGTFrmIni',[' '],'BusSettings',[' '])}
      mask init:
      | % blkh = gcbh;
      | % [sfi, sfp, sfpt] = rti_fpga_blockinitial(blkh,'UPDATEPARAMETER');
      | % rti_fpga_blockinitial(blkh,'UPDATEBLOCKGUI');
      settings: CopyFcn=try, rti_fpga_blk_copyfcn(gcbh); catch,errordlg({lasterr, '','Please check your RTI installation.'},['Error: ' upper(bdroot)], 'replace'); end  DeleteFcn=try, rti_fpga_blk_deletefcn(gcbh); catch,errordlg({lasterr, '','Please check your RTI installation.'},['Error: ' upper(bdroot)], 'replace'); end  ModelCloseFcn=try, rti_fpga_blk_modelclosefcn(gcbh); catch,errordlg({lasterr, '','Please check your RTI installation.'},['Error: ' upper(bdroot)], 'replace'); end  PreSaveFcn=try, rti_fpga_blk_presavefcn(gcbh); catch,errordlg({lasterr, '','Please check your RTI installation.'},['Error: ' upper(bdroot)], 'replace'); end  NameChangeFcn=try, rti_fpga_blk_namechangefcn(gcbh); catch,errordlg({lasterr, '','Please check your RTI installation.'},['Error: ' upper(bdroot)], 'replace'); end  OpenFcn=try, rti_fpga_blk_openfcn(gcbh); catch,errordlg({lasterr, '','Please check your RTI installation.'},['Error: ' upper(bdroot)], 'replace'); end  CloseFcn=try, rti_fpga_blk_closefcn(gcbh); catch,errordlg({lasterr, '','Please check your RTI installation.'},['Error: ' upper(bdroot)], 'replace'); end  ParentCloseFcn=try, rti_fpga_blk_parentclosefcn(gcbh); catch,errordlg({lasterr, '','Please check your RTI installation.'},['Error: ' upper(bdroot)], 'replace'); end
      mask Help: eval( ['lasterror(''reset''); rtifpgaguilib(''RTIMaskHelp'', gcbh);', 'disp(lasterr);']);
      mask Display: text(0.5,0.575,'Digital InOut 3 (Class 1)','HorizontalAlignment','center');text(0.5,0.425,'s3','HorizontalAlignment','center');
  FPGA_IO_WRITE_BL3 : Subsystem  LoadFcn=try, rti_fpga_blk_loadfcn(gcbh); catch,errordlg({lasterr, '','Please check your RTI installation.'},['Error: ' upper(bdroot)], 'replace'); end  InitFcn=try, rti_fpga_blk_initfcn(gcbh); catch,errordlg({lasterr, '','Please check your RTI installation.'},['Error: ' upper(bdroot)], 'replace'); end  StartFcn=try, rti_fpga_blk_startfcn(gcbh); catch,errordlg({lasterr, '','Please check your RTI installation.'},['Error: ' upper(bdroot)], 'replace'); end  mask(RTI){DSProperties=struct('RTI',struct('Version',uint32(6),'BlockType',struct('isSLSource',uint8(0),'isSLSink',uint8(0),'isHWSource',uint8(0),'isHWSink',uint8(0),'isSetup',uint8(1),'isInline',uint8(1),'isNonInline',uint8(0),'isInterrupt',uint8(0),'isChannelwise',uint8(0)),'IOBoardType','DSFPGA','UnitType','','Identifier','IOWRITE','DialogType','ML','BlockSet','FPGA','SlaveProcessor','')), RTIBlockInterface=struct('InputPortsActive',1,'InputPortsWidth',int32(1),'InputPortsDataType',{{'SS_DOUBLE'}},'InputPortsName',{{['To IO']}},'InitLevel',3,'DialogFcn','rtifpgaiowritegui','BlockDisplay',{{['FPGA IO Write'],'auto'}},'IconTransparency','on','BlockName',struct('Token',{{'FPGA_IO_Write_BL1'}})), RTIBlockParameters=struct('BoardNo',{{1,'OFF',[1 16]}},'IOType',{{'All','OFF',[]}},'ChannelNo',{{'4','OFF',[]}},'FrmIni',{{'fpga_framework_ini_DS1302_XC7K325T_FLEXIBLEIO','OFF',[]}},'IOFrmIni',{{'','OFF',[]}},'Name',{{['Digital InOut 4 (Class 1)'],'OFF',[]}},'DynFcn',{{struct('GUIPar',struct('Name',{{'Used'},{['Invert values']},{['Input filter (0ns..10,000,000ns)']},{['Input filter calculated']},{['High supply']},{['Rising edge delay (0ns..655350ns)']},{['Enable digital out simulation port']},{['Enable digital in simulation port']},{['Rising edge delay calculated']},{['Invert input polarity']},{['Invert output polarity']},{['Enable FPGA test access and scaling for this block']}},'GUIType',{{'none'},{'popup','Off','On'},{'edit'},{'none'},{'popup','5V','3.3V','2.5V'},{'edit'},{'checkbox'},{'checkbox'},{'none'},{'popup','Disabled','Enabled'},{'popup','Disabled','Enabled'},{'checkbox'}},'Range',{{'0','1'},{'0','1'},{''},{[0 1 2 3 4 5 6 7 8 9 10 11 12 13 14 15 16 17 18 19 20 21 22 23 24 25 26 27 28 29 30 31 32 33 34 35 36 37 38 39 40 41 42 43 44 45 46 47 48 49 50 51 52 53 54 55 56 57 58 59 60 61 62 63 64 65 66 67 68 69 70 71 72 73 74 75 76 77 78 79 80 81 82 83 84 85 86 87 88 89 90 91 92 93 94 95 96 97 98 99 100 101 102 103 104 105 106 107 108 109 110 111 112 113 114 115 116 117 118 119 120 121 122 123 124 125 126 127 128 129 130 131 132 133 134 135 136 137 138 139 140 141 142 143 144 145 146 147 148 149 150 151 152 153 154 155 156 157 158 159 160 161 162 163 164 165 166 167 168 169 170 171 172 173 174 175 176 177 178 179 180 181 182 183 184 185 186 187 188 189 190 191 192 193 194 195 196 197 198 199 200 201 202 203 204 205 206 207 208 209 210 211 212 213 214 215 216 217 218 219 220 221 222 223 224 225 226 227 228 229 230 231 232 233 234 235 236 237 238 239 240 241 242 243 244 245 246 247 248 249 250 251 252 253 254 255 256 257 258 259 260 261 262 263 264 265 266 267 268 269 270 271 272 273 274 275 276 277 278 279 280 281 282 283 284 285 286 287 288 289 290 291 292 293 294 295 296 297 298 299 300 301 302 303 304 305 306 307 308 309 310 311 312 313 314 315 316 317 318 319 320 321 322 323 324 325 326 327 328 329 330 331 332 333 334 335 336 337 338 339 340 341 342 343 344 345 346 347 348 349 350 351 352 353 354 355 356 357 358 359 360 361 362 363 364 365 366 367 368 369 370 371 372 373 374 375 376 377 378 379 380 381 382 383 384 385 386 387 388 389 390 391 392 393 394 395 396 397 398 399 400 401 402 403 404 405 406 407 408 409 410 411 412 413 414 415 416 417 418 419 420 421 422 423 424 425 426 427 428 429 430 431 432 433 434 435 436 437 438 439 440 441 442 443 444 445 446 447 448 449 450 451 452 453 454 455 456 457 458 459 460 461 462 463 464 465 466 467 468 469 470 471 472 473 474 475 476 477 478 479 480 481 482 483 484 485 486 487 488 489 490 491 492 493 494 495 496 497 498 499 500 501 502 503 504 505 506 507 508 509 510 511]},{'0','1','2'},{''},{'0','1'},{'0','1'},{[0 1 2 3 4 5 6 7 8 9 10 11 12 13 14 15 16 17 18 19 20 21 22 23 24 25 26 27 28 29 30 31 32 33 34 35 36 37 38 39 40 41 42 43 44 45 46 47 48 49 50 51 52 53 54 55 56 57 58 59 60 61 62 63 64 65 66 67 68 69 70 71 72 73 74 75 76 77 78 79 80 81 82 83 84 85 86 87 88 89 90 91 92 93 94 95 96 97 98 99 100 101 102 103 104 105 106 107 108 109 110 111 112 113 114 115 116 117 118 119 120 121 122 123 124 125 126 127 128 129 130 131 132 133 134 135 136 137 138 139 140 141 142 143 144 145 146 147 148 149 150 151 152 153 154 155 156 157 158 159 160 161 162 163 164 165 166 167 168 169 170 171 172 173 174 175 176 177 178 179 180 181 182 183 184 185 186 187 188 189 190 191 192 193 194 195 196 197 198 199 200 201 202 203 204 205 206 207 208 209 210 211 212 213 214 215 216 217 218 219 220 221 222 223 224 225 226 227 228 229 230 231 232 233 234 235 236 237 238 239 240 241 242 243 244 245 246 247 248 249 250 251 252 253 254 255 256 257 258 259 260 261 262 263 264 265 266 267 268 269 270 271 272 273 274 275 276 277 278 279 280 281 282 283 284 285 286 287 288 289 290 291 292 293 294 295 296 297 298 299 300 301 302 303 304 305 306 307 308 309 310 311 312 313 314 315 316 317 318 319 320 321 322 323 324 325 326 327 328 329 330 331 332 333 334 335 336 337 338 339 340 341 342 343 344 345 346 347 348 349 350 351 352 353 354 355 356 357 358 359 360 361 362 363 364 365 366 367 368 369 370 371 372 373 374 375 376 377 378 379 380 381 382 383 384 385 386 387 388 389 390 391 392 393 394 395 396 397 398 399 400 401 402 403 404 405 406 407 408 409 410 411 412 413 414 415 416 417 418 419 420 421 422 423 424 425 426 427 428 429 430 431 432 433 434 435 436 437 438 439 440 441 442 443 444 445 446 447 448 449 450 451 452 453 454 455 456 457 458 459 460 461 462 463 464 465 466 467 468 469 470 471 472 473 474 475 476 477 478 479 480 481 482 483 484 485 486 487 488 489 490 491 492 493 494 495 496 497 498 499 500 501 502 503 504 505 506 507 508 509 510 511 512 513 514 515 516 517 518 519 520 521 522 523 524 525 526 527 528 529 530 531 532 533 534 535 536 537 538 539 540 541 542 543 544 545 546 547 548 549 550 551 552 553 554 555 556 557 558 559 560 561 562 563 564 565 566 567 568 569 570 571 572 573 574 575 576 577 578 579 580 581 582 583 584 585 586 587 588 589 590 591 592 593 594 595 596 597 598 599 600 601 602 603 604 605 606 607 608 609 610 611 612 613 614 615 616 617 618 619 620 621 622 623 624 625 626 627 628 629 630 631 632 633 634 635 636 637 638 639 640 641 642 643 644 645 646 647 648 649 650 651 652 653 654 655 656 657 658 659 660 661 662 663 664 665 666 667 668 669 670 671 672 673 674 675 676 677 678 679 680 681 682 683 684 685 686 687 688 689 690 691 692 693 694 695 696 697 698 699 700 701 702 703 704 705 706 707 708 709 710 711 712 713 714 715 716 717 718 719 720 721 722 723 724 725 726 727 728 729 730 731 732 733 734 735 736 737 738 739 740 741 742 743 744 745 746 747 748 749 750 751 752 753 754 755 756 757 758 759 760 761 762 763 764 765 766 767 768 769 770 771 772 773 774 775 776 777 778 779 780 781 782 783 784 785 786 787 788 789 790 791 792 793 794 795 796 797 798 799 800 801 802 803 804 805 806 807 808 809 810 811 812 813 814 815 816 817 818 819 820 821 822 823 824 825 826 827 828 829 830 831 832 833 834 835 836 837 838 839 840 841 842 843 844 845 846 847 848 849 850 851 852 853 854 855 856 857 858 859 860 861 862 863 864 865 866 867 868 869 870 871 872 873 874 875 876 877 878 879 880 881 882 883 884 885 886 887 888 889 890 891 892 893 894 895 896 897 898 899 900 901 902 903 904 905 906 907 908 909 910 911 912 913 914 915 916 917 918 919 920 921 922 923 924 925 926 927 928 929 930 931 932 933 934 935 936 937 938 939 940 941 942 943 944 945 946 947 948 949 950 951 952 953 954 955 956 957 958 959 960 961 962 963 964 965 966 967 968 969 970 971 972 973 974 975 976 977 978 979 980 981 982 983 984 985 986 987 988 989 990 991 992 993 994 995 996 997 998 999 1000 1001 1002 1003 1004 1005 1006 1007 1008 1009 1010 1011 1012 1013 1014 1015 1016 1017 1018 1019 1020 ...(+378111 chars)]},{'0','1'},{'0','1'},{'0','1'}},'Init',{{'1','0'},{'0'},{'0'},{'0'},{'0'},{'0'},{'0'},{'0'},{'0'},{'0'},{'0'},{'1'}},'Group',{{''},{''},{''},{''},{''},{''},{''},{''},{''},{''},{''},{''}},'Generic',{{'diotp1_03_used'},{'diotp1_03_invert'},{'DIGINOUT_03FILTER'},{'diotp1_03_filter'},{'diotp1_03_voltage'},{'DIGINOUT_03_DELAY'},{''},{''},{'diotp1_03_delay'},{'RTIFPGA_INVERT_INPUT_POLARITY(03)'},{'RTIFPGA_INVERT_OUTPUT_POLARITY(03)'},{'RTIFPGA_TA_SCALING_ENABLE(03)'}},'Application',{{''},{''},{''},{''},{''},{''},{'ApplicationIn(2).Show'},{'ApplicationOut(4).Show'},{''},{''},{''},{''}},'Framework',{{''},{''},{''},{''},{''},{''},{''},{''},{''},{''},{''},{''}},'Callback',{{''},{''},{'fpga_framework_ini_DS1302_XC7K325T_FLEXIBLEIO:input_filter_calculation'},{''},{''},{'fpga_framework_ini_DS1302_XC7K325T_FLEXIBLEIO:rising_edge_delay_calculation'},{''},{''},{''},{''},{''},{''}},'Tab',{[],[],[],[],[],[],[],[],[],{'3'},{'3'},{'3'}},'Tag',{[],[],[],[],[],[],[],[],[],[],[],{''}}),'Exl',{{''}},'HlpFile',{{'rtifpga','DIGITAL_INOUT_CL1_DS1302'}},'Hlp',{{['Click below for further details on this I/O function.']}},'Gen',struct('name',{'diotp1_03_used','diotp1_03_invert','DIGINOUT_03FILTER','diotp1_03_filter','diotp1_03_voltage','DIGINOUT_03_DELAY','','','diotp1_03_delay','RTIFPGA_INVERT_INPUT_POLARITY(03)','RTIFPGA_INVERT_OUTPUT_POLARITY(03)','RTIFPGA_TA_SCALING_ENABLE(03)'},'value',{'1','0','0','0','0','0','','','0','0','0','1'},'unusedinit',{'0','','','','','','','','','','',''},'tag',{'','','','','','','','','','','',''},'filename',{'','','','','','','','','','','',''}),'Frm',struct('FrameworkOut',struct('Name',{{'diotp1_03_out'},{'diotp1_03_ena'},{'diotp1_03_dir'}},'BitWidth',{{'1'},{'1'},{'1'}},'BinaryPoint',{{'0'},{'0'},{'0'}},'Format',{{'unsigned'},{'unsigned'},{'unsigned'}},'Invert',{{'0'},[],[]},'RplcV',{{'0'},{'0'},{'0'}},'SwchV',{{'0'},{'0'},{'0'}}),'FrameworkIn',struct('Name',{{'diotp1_03_in'}},'BitWidth',{{'1'}},'BinaryPoint',{{'0'}},'Format',{{'unsigned'}},'Invert',{{'0'}},'RplcV',{{'0'}},'SwchV',{{'0'}})),'App',struct('ApplicationOut',struct('Name',{{['Data Out']},{'Enable'},{'Direction'},{['Sim Data In']}},'Show',{{true},{true},{true},{0}}),'ApplicationIn',struct('Name',{{['Data In']},{['Sim Data Out']}},'Show',{{true},{0}})),'Con',{{'FrameworkIn(1)','ApplicationIn(1)','FrameworkOut(1)','ApplicationOut(1)','FrameworkOut(2)','ApplicationOut(2)','FrameworkOut(3)','ApplicationOut(3)'}},'OffCon',{{'data_in_o','FrameworkIn(1)','data_in_i','ApplicationOut(4)','data_out_i','FrameworkOut(1)','data_out_o','ApplicationIn(2)','enable_i','FrameworkOut(2)','direction_i','FrameworkOut(3)'}},'OffModel',{{'dig_inout_tp1'}}),'OFF',[]}},'FPGAFrameworkId',{{'8','OFF',[]}},'CustomName',{{'s4','OFF',[]}},'MGTFrmIni',{{'','OFF',[]}},'BusSettings',{{[' '],'OFF',[]}}), RTISFcnParameters=struct('BoardNo','double'), RTIBlockParaDefault=struct('BoardNo',1,'IOType','All','ChannelNo',[' '],'FrmIni',[' '],'IOFrmIni',[' '],'Name',[' '],'DynFcn',struct('GUIPar','','Hlp','','HlpFile','','Exl','','Frm','','Gen','','App','','Con',''),'FPGAFrameworkId',[' '],'CustomName',[' '],'MGTFrmIni',[' '],'BusSettings',[' '])}
      mask init:
      | % blkh = gcbh;
      | % [sfi, sfp, sfpt] = rti_fpga_blockinitial(blkh,'UPDATEPARAMETER');
      | % rti_fpga_blockinitial(blkh,'UPDATEBLOCKGUI');
      settings: CopyFcn=try, rti_fpga_blk_copyfcn(gcbh); catch,errordlg({lasterr, '','Please check your RTI installation.'},['Error: ' upper(bdroot)], 'replace'); end  DeleteFcn=try, rti_fpga_blk_deletefcn(gcbh); catch,errordlg({lasterr, '','Please check your RTI installation.'},['Error: ' upper(bdroot)], 'replace'); end  ModelCloseFcn=try, rti_fpga_blk_modelclosefcn(gcbh); catch,errordlg({lasterr, '','Please check your RTI installation.'},['Error: ' upper(bdroot)], 'replace'); end  PreSaveFcn=try, rti_fpga_blk_presavefcn(gcbh); catch,errordlg({lasterr, '','Please check your RTI installation.'},['Error: ' upper(bdroot)], 'replace'); end  NameChangeFcn=try, rti_fpga_blk_namechangefcn(gcbh); catch,errordlg({lasterr, '','Please check your RTI installation.'},['Error: ' upper(bdroot)], 'replace'); end  OpenFcn=try, rti_fpga_blk_openfcn(gcbh); catch,errordlg({lasterr, '','Please check your RTI installation.'},['Error: ' upper(bdroot)], 'replace'); end  CloseFcn=try, rti_fpga_blk_closefcn(gcbh); catch,errordlg({lasterr, '','Please check your RTI installation.'},['Error: ' upper(bdroot)], 'replace'); end  ParentCloseFcn=try, rti_fpga_blk_parentclosefcn(gcbh); catch,errordlg({lasterr, '','Please check your RTI installation.'},['Error: ' upper(bdroot)], 'replace'); end
      mask Help: eval( ['lasterror(''reset''); rtifpgaguilib(''RTIMaskHelp'', gcbh);', 'disp(lasterr);']);
      mask Display: text(0.5,0.575,'Digital InOut 4 (Class 1)','HorizontalAlignment','center');text(0.5,0.425,'s4','HorizontalAlignment','center');
  FPGA_IO_WRITE_BL4 : Subsystem  LoadFcn=try, rti_fpga_blk_loadfcn(gcbh); catch,errordlg({lasterr, '','Please check your RTI installation.'},['Error: ' upper(bdroot)], 'replace'); end  InitFcn=try, rti_fpga_blk_initfcn(gcbh); catch,errordlg({lasterr, '','Please check your RTI installation.'},['Error: ' upper(bdroot)], 'replace'); end  StartFcn=try, rti_fpga_blk_startfcn(gcbh); catch,errordlg({lasterr, '','Please check your RTI installation.'},['Error: ' upper(bdroot)], 'replace'); end  mask(RTI){DSProperties=struct('RTI',struct('Version',uint32(6),'BlockType',struct('isSLSource',uint8(0),'isSLSink',uint8(0),'isHWSource',uint8(0),'isHWSink',uint8(0),'isSetup',uint8(1),'isInline',uint8(1),'isNonInline',uint8(0),'isInterrupt',uint8(0),'isChannelwise',uint8(0)),'IOBoardType','DSFPGA','UnitType','','Identifier','IOWRITE','DialogType','ML','BlockSet','FPGA','SlaveProcessor','')), RTIBlockInterface=struct('InputPortsActive',1,'InputPortsWidth',int32(1),'InputPortsDataType',{{'SS_DOUBLE'}},'InputPortsName',{{['To IO']}},'InitLevel',3,'DialogFcn','rtifpgaiowritegui','BlockDisplay',{{['FPGA IO Write'],'auto'}},'IconTransparency','on','BlockName',struct('Token',{{'FPGA_IO_Write_BL1'}})), RTIBlockParameters=struct('BoardNo',{{1,'OFF',[1 16]}},'IOType',{{'All','OFF',[]}},'ChannelNo',{{'5','OFF',[]}},'FrmIni',{{'fpga_framework_ini_DS1302_XC7K325T_FLEXIBLEIO','OFF',[]}},'IOFrmIni',{{'','OFF',[]}},'Name',{{['Digital InOut 5 (Class 1)'],'OFF',[]}},'DynFcn',{{struct('GUIPar',struct('Name',{{'Used'},{['Invert values']},{['Input filter (0ns..10,000,000ns)']},{['Input filter calculated']},{['High supply']},{['Rising edge delay (0ns..655350ns)']},{['Enable digital out simulation port']},{['Enable digital in simulation port']},{['Rising edge delay calculated']},{['Invert input polarity']},{['Invert output polarity']},{['Enable FPGA test access and scaling for this block']}},'GUIType',{{'none'},{'popup','Off','On'},{'edit'},{'none'},{'popup','5V','3.3V','2.5V'},{'edit'},{'checkbox'},{'checkbox'},{'none'},{'popup','Disabled','Enabled'},{'popup','Disabled','Enabled'},{'checkbox'}},'Range',{{'0','1'},{'0','1'},{''},{[0 1 2 3 4 5 6 7 8 9 10 11 12 13 14 15 16 17 18 19 20 21 22 23 24 25 26 27 28 29 30 31 32 33 34 35 36 37 38 39 40 41 42 43 44 45 46 47 48 49 50 51 52 53 54 55 56 57 58 59 60 61 62 63 64 65 66 67 68 69 70 71 72 73 74 75 76 77 78 79 80 81 82 83 84 85 86 87 88 89 90 91 92 93 94 95 96 97 98 99 100 101 102 103 104 105 106 107 108 109 110 111 112 113 114 115 116 117 118 119 120 121 122 123 124 125 126 127 128 129 130 131 132 133 134 135 136 137 138 139 140 141 142 143 144 145 146 147 148 149 150 151 152 153 154 155 156 157 158 159 160 161 162 163 164 165 166 167 168 169 170 171 172 173 174 175 176 177 178 179 180 181 182 183 184 185 186 187 188 189 190 191 192 193 194 195 196 197 198 199 200 201 202 203 204 205 206 207 208 209 210 211 212 213 214 215 216 217 218 219 220 221 222 223 224 225 226 227 228 229 230 231 232 233 234 235 236 237 238 239 240 241 242 243 244 245 246 247 248 249 250 251 252 253 254 255 256 257 258 259 260 261 262 263 264 265 266 267 268 269 270 271 272 273 274 275 276 277 278 279 280 281 282 283 284 285 286 287 288 289 290 291 292 293 294 295 296 297 298 299 300 301 302 303 304 305 306 307 308 309 310 311 312 313 314 315 316 317 318 319 320 321 322 323 324 325 326 327 328 329 330 331 332 333 334 335 336 337 338 339 340 341 342 343 344 345 346 347 348 349 350 351 352 353 354 355 356 357 358 359 360 361 362 363 364 365 366 367 368 369 370 371 372 373 374 375 376 377 378 379 380 381 382 383 384 385 386 387 388 389 390 391 392 393 394 395 396 397 398 399 400 401 402 403 404 405 406 407 408 409 410 411 412 413 414 415 416 417 418 419 420 421 422 423 424 425 426 427 428 429 430 431 432 433 434 435 436 437 438 439 440 441 442 443 444 445 446 447 448 449 450 451 452 453 454 455 456 457 458 459 460 461 462 463 464 465 466 467 468 469 470 471 472 473 474 475 476 477 478 479 480 481 482 483 484 485 486 487 488 489 490 491 492 493 494 495 496 497 498 499 500 501 502 503 504 505 506 507 508 509 510 511]},{'0','1','2'},{''},{'0','1'},{'0','1'},{[0 1 2 3 4 5 6 7 8 9 10 11 12 13 14 15 16 17 18 19 20 21 22 23 24 25 26 27 28 29 30 31 32 33 34 35 36 37 38 39 40 41 42 43 44 45 46 47 48 49 50 51 52 53 54 55 56 57 58 59 60 61 62 63 64 65 66 67 68 69 70 71 72 73 74 75 76 77 78 79 80 81 82 83 84 85 86 87 88 89 90 91 92 93 94 95 96 97 98 99 100 101 102 103 104 105 106 107 108 109 110 111 112 113 114 115 116 117 118 119 120 121 122 123 124 125 126 127 128 129 130 131 132 133 134 135 136 137 138 139 140 141 142 143 144 145 146 147 148 149 150 151 152 153 154 155 156 157 158 159 160 161 162 163 164 165 166 167 168 169 170 171 172 173 174 175 176 177 178 179 180 181 182 183 184 185 186 187 188 189 190 191 192 193 194 195 196 197 198 199 200 201 202 203 204 205 206 207 208 209 210 211 212 213 214 215 216 217 218 219 220 221 222 223 224 225 226 227 228 229 230 231 232 233 234 235 236 237 238 239 240 241 242 243 244 245 246 247 248 249 250 251 252 253 254 255 256 257 258 259 260 261 262 263 264 265 266 267 268 269 270 271 272 273 274 275 276 277 278 279 280 281 282 283 284 285 286 287 288 289 290 291 292 293 294 295 296 297 298 299 300 301 302 303 304 305 306 307 308 309 310 311 312 313 314 315 316 317 318 319 320 321 322 323 324 325 326 327 328 329 330 331 332 333 334 335 336 337 338 339 340 341 342 343 344 345 346 347 348 349 350 351 352 353 354 355 356 357 358 359 360 361 362 363 364 365 366 367 368 369 370 371 372 373 374 375 376 377 378 379 380 381 382 383 384 385 386 387 388 389 390 391 392 393 394 395 396 397 398 399 400 401 402 403 404 405 406 407 408 409 410 411 412 413 414 415 416 417 418 419 420 421 422 423 424 425 426 427 428 429 430 431 432 433 434 435 436 437 438 439 440 441 442 443 444 445 446 447 448 449 450 451 452 453 454 455 456 457 458 459 460 461 462 463 464 465 466 467 468 469 470 471 472 473 474 475 476 477 478 479 480 481 482 483 484 485 486 487 488 489 490 491 492 493 494 495 496 497 498 499 500 501 502 503 504 505 506 507 508 509 510 511 512 513 514 515 516 517 518 519 520 521 522 523 524 525 526 527 528 529 530 531 532 533 534 535 536 537 538 539 540 541 542 543 544 545 546 547 548 549 550 551 552 553 554 555 556 557 558 559 560 561 562 563 564 565 566 567 568 569 570 571 572 573 574 575 576 577 578 579 580 581 582 583 584 585 586 587 588 589 590 591 592 593 594 595 596 597 598 599 600 601 602 603 604 605 606 607 608 609 610 611 612 613 614 615 616 617 618 619 620 621 622 623 624 625 626 627 628 629 630 631 632 633 634 635 636 637 638 639 640 641 642 643 644 645 646 647 648 649 650 651 652 653 654 655 656 657 658 659 660 661 662 663 664 665 666 667 668 669 670 671 672 673 674 675 676 677 678 679 680 681 682 683 684 685 686 687 688 689 690 691 692 693 694 695 696 697 698 699 700 701 702 703 704 705 706 707 708 709 710 711 712 713 714 715 716 717 718 719 720 721 722 723 724 725 726 727 728 729 730 731 732 733 734 735 736 737 738 739 740 741 742 743 744 745 746 747 748 749 750 751 752 753 754 755 756 757 758 759 760 761 762 763 764 765 766 767 768 769 770 771 772 773 774 775 776 777 778 779 780 781 782 783 784 785 786 787 788 789 790 791 792 793 794 795 796 797 798 799 800 801 802 803 804 805 806 807 808 809 810 811 812 813 814 815 816 817 818 819 820 821 822 823 824 825 826 827 828 829 830 831 832 833 834 835 836 837 838 839 840 841 842 843 844 845 846 847 848 849 850 851 852 853 854 855 856 857 858 859 860 861 862 863 864 865 866 867 868 869 870 871 872 873 874 875 876 877 878 879 880 881 882 883 884 885 886 887 888 889 890 891 892 893 894 895 896 897 898 899 900 901 902 903 904 905 906 907 908 909 910 911 912 913 914 915 916 917 918 919 920 921 922 923 924 925 926 927 928 929 930 931 932 933 934 935 936 937 938 939 940 941 942 943 944 945 946 947 948 949 950 951 952 953 954 955 956 957 958 959 960 961 962 963 964 965 966 967 968 969 970 971 972 973 974 975 976 977 978 979 980 981 982 983 984 985 986 987 988 989 990 991 992 993 994 995 996 997 998 999 1000 1001 1002 1003 1004 1005 1006 1007 1008 1009 1010 1011 1012 1013 1014 1015 1016 1017 1018 1019 1020 ...(+378111 chars)]},{'0','1'},{'0','1'},{'0','1'}},'Init',{{'1','0'},{'0'},{'0'},{'0'},{'0'},{'0'},{'0'},{'0'},{'0'},{'0'},{'0'},{'1'}},'Group',{{''},{''},{''},{''},{''},{''},{''},{''},{''},{''},{''},{''}},'Generic',{{'diotp1_04_used'},{'diotp1_04_invert'},{'DIGINOUT_04FILTER'},{'diotp1_04_filter'},{'diotp1_04_voltage'},{'DIGINOUT_04_DELAY'},{''},{''},{'diotp1_04_delay'},{'RTIFPGA_INVERT_INPUT_POLARITY(04)'},{'RTIFPGA_INVERT_OUTPUT_POLARITY(04)'},{'RTIFPGA_TA_SCALING_ENABLE(04)'}},'Application',{{''},{''},{''},{''},{''},{''},{'ApplicationIn(2).Show'},{'ApplicationOut(4).Show'},{''},{''},{''},{''}},'Framework',{{''},{''},{''},{''},{''},{''},{''},{''},{''},{''},{''},{''}},'Callback',{{''},{''},{'fpga_framework_ini_DS1302_XC7K325T_FLEXIBLEIO:input_filter_calculation'},{''},{''},{'fpga_framework_ini_DS1302_XC7K325T_FLEXIBLEIO:rising_edge_delay_calculation'},{''},{''},{''},{''},{''},{''}},'Tab',{[],[],[],[],[],[],[],[],[],{'3'},{'3'},{'3'}},'Tag',{[],[],[],[],[],[],[],[],[],[],[],{''}}),'Exl',{{''}},'HlpFile',{{'rtifpga','DIGITAL_INOUT_CL1_DS1302'}},'Hlp',{{['Click below for further details on this I/O function.']}},'Gen',struct('name',{'diotp1_04_used','diotp1_04_invert','DIGINOUT_04FILTER','diotp1_04_filter','diotp1_04_voltage','DIGINOUT_04_DELAY','','','diotp1_04_delay','RTIFPGA_INVERT_INPUT_POLARITY(04)','RTIFPGA_INVERT_OUTPUT_POLARITY(04)','RTIFPGA_TA_SCALING_ENABLE(04)'},'value',{'1','0','0','0','0','0','','','0','0','0','1'},'unusedinit',{'0','','','','','','','','','','',''},'tag',{'','','','','','','','','','','',''},'filename',{'','','','','','','','','','','',''}),'Frm',struct('FrameworkOut',struct('Name',{{'diotp1_04_out'},{'diotp1_04_ena'},{'diotp1_04_dir'}},'BitWidth',{{'1'},{'1'},{'1'}},'BinaryPoint',{{'0'},{'0'},{'0'}},'Format',{{'unsigned'},{'unsigned'},{'unsigned'}},'Invert',{{'0'},[],[]},'RplcV',{{'0'},{'0'},{'0'}},'SwchV',{{'0'},{'0'},{'0'}}),'FrameworkIn',struct('Name',{{'diotp1_04_in'}},'BitWidth',{{'1'}},'BinaryPoint',{{'0'}},'Format',{{'unsigned'}},'Invert',{{'0'}},'RplcV',{{'0'}},'SwchV',{{'0'}})),'App',struct('ApplicationOut',struct('Name',{{['Data Out']},{'Enable'},{'Direction'},{['Sim Data In']}},'Show',{{true},{true},{true},{0}}),'ApplicationIn',struct('Name',{{['Data In']},{['Sim Data Out']}},'Show',{{true},{0}})),'Con',{{'FrameworkIn(1)','ApplicationIn(1)','FrameworkOut(1)','ApplicationOut(1)','FrameworkOut(2)','ApplicationOut(2)','FrameworkOut(3)','ApplicationOut(3)'}},'OffCon',{{'data_in_o','FrameworkIn(1)','data_in_i','ApplicationOut(4)','data_out_i','FrameworkOut(1)','data_out_o','ApplicationIn(2)','enable_i','FrameworkOut(2)','direction_i','FrameworkOut(3)'}},'OffModel',{{'dig_inout_tp1'}}),'OFF',[]}},'FPGAFrameworkId',{{'8','OFF',[]}},'CustomName',{{'s5','OFF',[]}},'MGTFrmIni',{{'','OFF',[]}},'BusSettings',{{[' '],'OFF',[]}}), RTISFcnParameters=struct('BoardNo','double'), RTIBlockParaDefault=struct('BoardNo',1,'IOType','All','ChannelNo',[' '],'FrmIni',[' '],'IOFrmIni',[' '],'Name',[' '],'DynFcn',struct('GUIPar','','Hlp','','HlpFile','','Exl','','Frm','','Gen','','App','','Con',''),'FPGAFrameworkId',[' '],'CustomName',[' '],'MGTFrmIni',[' '],'BusSettings',[' '])}
      mask init:
      | % blkh = gcbh;
      | % [sfi, sfp, sfpt] = rti_fpga_blockinitial(blkh,'UPDATEPARAMETER');
      | % rti_fpga_blockinitial(blkh,'UPDATEBLOCKGUI');
      settings: CopyFcn=try, rti_fpga_blk_copyfcn(gcbh); catch,errordlg({lasterr, '','Please check your RTI installation.'},['Error: ' upper(bdroot)], 'replace'); end  DeleteFcn=try, rti_fpga_blk_deletefcn(gcbh); catch,errordlg({lasterr, '','Please check your RTI installation.'},['Error: ' upper(bdroot)], 'replace'); end  ModelCloseFcn=try, rti_fpga_blk_modelclosefcn(gcbh); catch,errordlg({lasterr, '','Please check your RTI installation.'},['Error: ' upper(bdroot)], 'replace'); end  PreSaveFcn=try, rti_fpga_blk_presavefcn(gcbh); catch,errordlg({lasterr, '','Please check your RTI installation.'},['Error: ' upper(bdroot)], 'replace'); end  NameChangeFcn=try, rti_fpga_blk_namechangefcn(gcbh); catch,errordlg({lasterr, '','Please check your RTI installation.'},['Error: ' upper(bdroot)], 'replace'); end  OpenFcn=try, rti_fpga_blk_openfcn(gcbh); catch,errordlg({lasterr, '','Please check your RTI installation.'},['Error: ' upper(bdroot)], 'replace'); end  CloseFcn=try, rti_fpga_blk_closefcn(gcbh); catch,errordlg({lasterr, '','Please check your RTI installation.'},['Error: ' upper(bdroot)], 'replace'); end  ParentCloseFcn=try, rti_fpga_blk_parentclosefcn(gcbh); catch,errordlg({lasterr, '','Please check your RTI installation.'},['Error: ' upper(bdroot)], 'replace'); end
      mask Help: eval( ['lasterror(''reset''); rtifpgaguilib(''RTIMaskHelp'', gcbh);', 'disp(lasterr);']);
      mask Display: text(0.5,0.575,'Digital InOut 5 (Class 1)','HorizontalAlignment','center');text(0.5,0.425,'s5','HorizontalAlignment','center');
  FPGA_IO_WRITE_BL5 : Subsystem  LoadFcn=try, rti_fpga_blk_loadfcn(gcbh); catch,errordlg({lasterr, '','Please check your RTI installation.'},['Error: ' upper(bdroot)], 'replace'); end  InitFcn=try, rti_fpga_blk_initfcn(gcbh); catch,errordlg({lasterr, '','Please check your RTI installation.'},['Error: ' upper(bdroot)], 'replace'); end  StartFcn=try, rti_fpga_blk_startfcn(gcbh); catch,errordlg({lasterr, '','Please check your RTI installation.'},['Error: ' upper(bdroot)], 'replace'); end  mask(RTI){DSProperties=struct('RTI',struct('Version',uint32(6),'BlockType',struct('isSLSource',uint8(0),'isSLSink',uint8(0),'isHWSource',uint8(0),'isHWSink',uint8(0),'isSetup',uint8(1),'isInline',uint8(1),'isNonInline',uint8(0),'isInterrupt',uint8(0),'isChannelwise',uint8(0)),'IOBoardType','DSFPGA','UnitType','','Identifier','IOWRITE','DialogType','ML','BlockSet','FPGA','SlaveProcessor','')), RTIBlockInterface=struct('InputPortsActive',1,'InputPortsWidth',int32(1),'InputPortsDataType',{{'SS_DOUBLE'}},'InputPortsName',{{['To IO']}},'InitLevel',3,'DialogFcn','rtifpgaiowritegui','BlockDisplay',{{['FPGA IO Write'],'auto'}},'IconTransparency','on','BlockName',struct('Token',{{'FPGA_IO_Write_BL1'}})), RTIBlockParameters=struct('BoardNo',{{1,'OFF',[1 16]}},'IOType',{{'All','OFF',[]}},'ChannelNo',{{'6','OFF',[]}},'FrmIni',{{'fpga_framework_ini_DS1302_XC7K325T_FLEXIBLEIO','OFF',[]}},'IOFrmIni',{{'','OFF',[]}},'Name',{{['Digital InOut 6 (Class 1)'],'OFF',[]}},'DynFcn',{{struct('GUIPar',struct('Name',{{'Used'},{['Invert values']},{['Input filter (0ns..10,000,000ns)']},{['Input filter calculated']},{['High supply']},{['Rising edge delay (0ns..655350ns)']},{['Enable digital out simulation port']},{['Enable digital in simulation port']},{['Rising edge delay calculated']},{['Invert input polarity']},{['Invert output polarity']},{['Enable FPGA test access and scaling for this block']}},'GUIType',{{'none'},{'popup','Off','On'},{'edit'},{'none'},{'popup','5V','3.3V','2.5V'},{'edit'},{'checkbox'},{'checkbox'},{'none'},{'popup','Disabled','Enabled'},{'popup','Disabled','Enabled'},{'checkbox'}},'Range',{{'0','1'},{'0','1'},{''},{[0 1 2 3 4 5 6 7 8 9 10 11 12 13 14 15 16 17 18 19 20 21 22 23 24 25 26 27 28 29 30 31 32 33 34 35 36 37 38 39 40 41 42 43 44 45 46 47 48 49 50 51 52 53 54 55 56 57 58 59 60 61 62 63 64 65 66 67 68 69 70 71 72 73 74 75 76 77 78 79 80 81 82 83 84 85 86 87 88 89 90 91 92 93 94 95 96 97 98 99 100 101 102 103 104 105 106 107 108 109 110 111 112 113 114 115 116 117 118 119 120 121 122 123 124 125 126 127 128 129 130 131 132 133 134 135 136 137 138 139 140 141 142 143 144 145 146 147 148 149 150 151 152 153 154 155 156 157 158 159 160 161 162 163 164 165 166 167 168 169 170 171 172 173 174 175 176 177 178 179 180 181 182 183 184 185 186 187 188 189 190 191 192 193 194 195 196 197 198 199 200 201 202 203 204 205 206 207 208 209 210 211 212 213 214 215 216 217 218 219 220 221 222 223 224 225 226 227 228 229 230 231 232 233 234 235 236 237 238 239 240 241 242 243 244 245 246 247 248 249 250 251 252 253 254 255 256 257 258 259 260 261 262 263 264 265 266 267 268 269 270 271 272 273 274 275 276 277 278 279 280 281 282 283 284 285 286 287 288 289 290 291 292 293 294 295 296 297 298 299 300 301 302 303 304 305 306 307 308 309 310 311 312 313 314 315 316 317 318 319 320 321 322 323 324 325 326 327 328 329 330 331 332 333 334 335 336 337 338 339 340 341 342 343 344 345 346 347 348 349 350 351 352 353 354 355 356 357 358 359 360 361 362 363 364 365 366 367 368 369 370 371 372 373 374 375 376 377 378 379 380 381 382 383 384 385 386 387 388 389 390 391 392 393 394 395 396 397 398 399 400 401 402 403 404 405 406 407 408 409 410 411 412 413 414 415 416 417 418 419 420 421 422 423 424 425 426 427 428 429 430 431 432 433 434 435 436 437 438 439 440 441 442 443 444 445 446 447 448 449 450 451 452 453 454 455 456 457 458 459 460 461 462 463 464 465 466 467 468 469 470 471 472 473 474 475 476 477 478 479 480 481 482 483 484 485 486 487 488 489 490 491 492 493 494 495 496 497 498 499 500 501 502 503 504 505 506 507 508 509 510 511]},{'0','1','2'},{''},{'0','1'},{'0','1'},{[0 1 2 3 4 5 6 7 8 9 10 11 12 13 14 15 16 17 18 19 20 21 22 23 24 25 26 27 28 29 30 31 32 33 34 35 36 37 38 39 40 41 42 43 44 45 46 47 48 49 50 51 52 53 54 55 56 57 58 59 60 61 62 63 64 65 66 67 68 69 70 71 72 73 74 75 76 77 78 79 80 81 82 83 84 85 86 87 88 89 90 91 92 93 94 95 96 97 98 99 100 101 102 103 104 105 106 107 108 109 110 111 112 113 114 115 116 117 118 119 120 121 122 123 124 125 126 127 128 129 130 131 132 133 134 135 136 137 138 139 140 141 142 143 144 145 146 147 148 149 150 151 152 153 154 155 156 157 158 159 160 161 162 163 164 165 166 167 168 169 170 171 172 173 174 175 176 177 178 179 180 181 182 183 184 185 186 187 188 189 190 191 192 193 194 195 196 197 198 199 200 201 202 203 204 205 206 207 208 209 210 211 212 213 214 215 216 217 218 219 220 221 222 223 224 225 226 227 228 229 230 231 232 233 234 235 236 237 238 239 240 241 242 243 244 245 246 247 248 249 250 251 252 253 254 255 256 257 258 259 260 261 262 263 264 265 266 267 268 269 270 271 272 273 274 275 276 277 278 279 280 281 282 283 284 285 286 287 288 289 290 291 292 293 294 295 296 297 298 299 300 301 302 303 304 305 306 307 308 309 310 311 312 313 314 315 316 317 318 319 320 321 322 323 324 325 326 327 328 329 330 331 332 333 334 335 336 337 338 339 340 341 342 343 344 345 346 347 348 349 350 351 352 353 354 355 356 357 358 359 360 361 362 363 364 365 366 367 368 369 370 371 372 373 374 375 376 377 378 379 380 381 382 383 384 385 386 387 388 389 390 391 392 393 394 395 396 397 398 399 400 401 402 403 404 405 406 407 408 409 410 411 412 413 414 415 416 417 418 419 420 421 422 423 424 425 426 427 428 429 430 431 432 433 434 435 436 437 438 439 440 441 442 443 444 445 446 447 448 449 450 451 452 453 454 455 456 457 458 459 460 461 462 463 464 465 466 467 468 469 470 471 472 473 474 475 476 477 478 479 480 481 482 483 484 485 486 487 488 489 490 491 492 493 494 495 496 497 498 499 500 501 502 503 504 505 506 507 508 509 510 511 512 513 514 515 516 517 518 519 520 521 522 523 524 525 526 527 528 529 530 531 532 533 534 535 536 537 538 539 540 541 542 543 544 545 546 547 548 549 550 551 552 553 554 555 556 557 558 559 560 561 562 563 564 565 566 567 568 569 570 571 572 573 574 575 576 577 578 579 580 581 582 583 584 585 586 587 588 589 590 591 592 593 594 595 596 597 598 599 600 601 602 603 604 605 606 607 608 609 610 611 612 613 614 615 616 617 618 619 620 621 622 623 624 625 626 627 628 629 630 631 632 633 634 635 636 637 638 639 640 641 642 643 644 645 646 647 648 649 650 651 652 653 654 655 656 657 658 659 660 661 662 663 664 665 666 667 668 669 670 671 672 673 674 675 676 677 678 679 680 681 682 683 684 685 686 687 688 689 690 691 692 693 694 695 696 697 698 699 700 701 702 703 704 705 706 707 708 709 710 711 712 713 714 715 716 717 718 719 720 721 722 723 724 725 726 727 728 729 730 731 732 733 734 735 736 737 738 739 740 741 742 743 744 745 746 747 748 749 750 751 752 753 754 755 756 757 758 759 760 761 762 763 764 765 766 767 768 769 770 771 772 773 774 775 776 777 778 779 780 781 782 783 784 785 786 787 788 789 790 791 792 793 794 795 796 797 798 799 800 801 802 803 804 805 806 807 808 809 810 811 812 813 814 815 816 817 818 819 820 821 822 823 824 825 826 827 828 829 830 831 832 833 834 835 836 837 838 839 840 841 842 843 844 845 846 847 848 849 850 851 852 853 854 855 856 857 858 859 860 861 862 863 864 865 866 867 868 869 870 871 872 873 874 875 876 877 878 879 880 881 882 883 884 885 886 887 888 889 890 891 892 893 894 895 896 897 898 899 900 901 902 903 904 905 906 907 908 909 910 911 912 913 914 915 916 917 918 919 920 921 922 923 924 925 926 927 928 929 930 931 932 933 934 935 936 937 938 939 940 941 942 943 944 945 946 947 948 949 950 951 952 953 954 955 956 957 958 959 960 961 962 963 964 965 966 967 968 969 970 971 972 973 974 975 976 977 978 979 980 981 982 983 984 985 986 987 988 989 990 991 992 993 994 995 996 997 998 999 1000 1001 1002 1003 1004 1005 1006 1007 1008 1009 1010 1011 1012 1013 1014 1015 1016 1017 1018 1019 1020 ...(+378111 chars)]},{'0','1'},{'0','1'},{'0','1'}},'Init',{{'1','0'},{'0'},{'0'},{'0'},{'0'},{'0'},{'0'},{'0'},{'0'},{'0'},{'0'},{'1'}},'Group',{{''},{''},{''},{''},{''},{''},{''},{''},{''},{''},{''},{''}},'Generic',{{'diotp1_05_used'},{'diotp1_05_invert'},{'DIGINOUT_05FILTER'},{'diotp1_05_filter'},{'diotp1_05_voltage'},{'DIGINOUT_05_DELAY'},{''},{''},{'diotp1_05_delay'},{'RTIFPGA_INVERT_INPUT_POLARITY(05)'},{'RTIFPGA_INVERT_OUTPUT_POLARITY(05)'},{'RTIFPGA_TA_SCALING_ENABLE(05)'}},'Application',{{''},{''},{''},{''},{''},{''},{'ApplicationIn(2).Show'},{'ApplicationOut(4).Show'},{''},{''},{''},{''}},'Framework',{{''},{''},{''},{''},{''},{''},{''},{''},{''},{''},{''},{''}},'Callback',{{''},{''},{'fpga_framework_ini_DS1302_XC7K325T_FLEXIBLEIO:input_filter_calculation'},{''},{''},{'fpga_framework_ini_DS1302_XC7K325T_FLEXIBLEIO:rising_edge_delay_calculation'},{''},{''},{''},{''},{''},{''}},'Tab',{[],[],[],[],[],[],[],[],[],{'3'},{'3'},{'3'}},'Tag',{[],[],[],[],[],[],[],[],[],[],[],{''}}),'Exl',{{''}},'HlpFile',{{'rtifpga','DIGITAL_INOUT_CL1_DS1302'}},'Hlp',{{['Click below for further details on this I/O function.']}},'Gen',struct('name',{'diotp1_05_used','diotp1_05_invert','DIGINOUT_05FILTER','diotp1_05_filter','diotp1_05_voltage','DIGINOUT_05_DELAY','','','diotp1_05_delay','RTIFPGA_INVERT_INPUT_POLARITY(05)','RTIFPGA_INVERT_OUTPUT_POLARITY(05)','RTIFPGA_TA_SCALING_ENABLE(05)'},'value',{'1','0','0','0','0','0','','','0','0','0','1'},'unusedinit',{'0','','','','','','','','','','',''},'tag',{'','','','','','','','','','','',''},'filename',{'','','','','','','','','','','',''}),'Frm',struct('FrameworkOut',struct('Name',{{'diotp1_05_out'},{'diotp1_05_ena'},{'diotp1_05_dir'}},'BitWidth',{{'1'},{'1'},{'1'}},'BinaryPoint',{{'0'},{'0'},{'0'}},'Format',{{'unsigned'},{'unsigned'},{'unsigned'}},'Invert',{{'0'},[],[]},'RplcV',{{'0'},{'0'},{'0'}},'SwchV',{{'0'},{'0'},{'0'}}),'FrameworkIn',struct('Name',{{'diotp1_05_in'}},'BitWidth',{{'1'}},'BinaryPoint',{{'0'}},'Format',{{'unsigned'}},'Invert',{{'0'}},'RplcV',{{'0'}},'SwchV',{{'0'}})),'App',struct('ApplicationOut',struct('Name',{{['Data Out']},{'Enable'},{'Direction'},{['Sim Data In']}},'Show',{{true},{true},{true},{0}}),'ApplicationIn',struct('Name',{{['Data In']},{['Sim Data Out']}},'Show',{{true},{0}})),'Con',{{'FrameworkIn(1)','ApplicationIn(1)','FrameworkOut(1)','ApplicationOut(1)','FrameworkOut(2)','ApplicationOut(2)','FrameworkOut(3)','ApplicationOut(3)'}},'OffCon',{{'data_in_o','FrameworkIn(1)','data_in_i','ApplicationOut(4)','data_out_i','FrameworkOut(1)','data_out_o','ApplicationIn(2)','enable_i','FrameworkOut(2)','direction_i','FrameworkOut(3)'}},'OffModel',{{'dig_inout_tp1'}}),'OFF',[]}},'FPGAFrameworkId',{{'8','OFF',[]}},'CustomName',{{['s6 '],'OFF',[]}},'MGTFrmIni',{{'','OFF',[]}},'BusSettings',{{[' '],'OFF',[]}}), RTISFcnParameters=struct('BoardNo','double'), RTIBlockParaDefault=struct('BoardNo',1,'IOType','All','ChannelNo',[' '],'FrmIni',[' '],'IOFrmIni',[' '],'Name',[' '],'DynFcn',struct('GUIPar','','Hlp','','HlpFile','','Exl','','Frm','','Gen','','App','','Con',''),'FPGAFrameworkId',[' '],'CustomName',[' '],'MGTFrmIni',[' '],'BusSettings',[' '])}
      mask init:
      | % blkh = gcbh;
      | % [sfi, sfp, sfpt] = rti_fpga_blockinitial(blkh,'UPDATEPARAMETER');
      | % rti_fpga_blockinitial(blkh,'UPDATEBLOCKGUI');
      settings: CopyFcn=try, rti_fpga_blk_copyfcn(gcbh); catch,errordlg({lasterr, '','Please check your RTI installation.'},['Error: ' upper(bdroot)], 'replace'); end  DeleteFcn=try, rti_fpga_blk_deletefcn(gcbh); catch,errordlg({lasterr, '','Please check your RTI installation.'},['Error: ' upper(bdroot)], 'replace'); end  ModelCloseFcn=try, rti_fpga_blk_modelclosefcn(gcbh); catch,errordlg({lasterr, '','Please check your RTI installation.'},['Error: ' upper(bdroot)], 'replace'); end  PreSaveFcn=try, rti_fpga_blk_presavefcn(gcbh); catch,errordlg({lasterr, '','Please check your RTI installation.'},['Error: ' upper(bdroot)], 'replace'); end  NameChangeFcn=try, rti_fpga_blk_namechangefcn(gcbh); catch,errordlg({lasterr, '','Please check your RTI installation.'},['Error: ' upper(bdroot)], 'replace'); end  OpenFcn=try, rti_fpga_blk_openfcn(gcbh); catch,errordlg({lasterr, '','Please check your RTI installation.'},['Error: ' upper(bdroot)], 'replace'); end  CloseFcn=try, rti_fpga_blk_closefcn(gcbh); catch,errordlg({lasterr, '','Please check your RTI installation.'},['Error: ' upper(bdroot)], 'replace'); end  ParentCloseFcn=try, rti_fpga_blk_parentclosefcn(gcbh); catch,errordlg({lasterr, '','Please check your RTI installation.'},['Error: ' upper(bdroot)], 'replace'); end
      mask Help: eval( ['lasterror(''reset''); rtifpgaguilib(''RTIMaskHelp'', gcbh);', 'disp(lasterr);']);
      mask Display: text(0.5,0.575,'Digital InOut 6 (Class 1)','HorizontalAlignment','center');text(0.5,0.425,'s6 ','HorizontalAlignment','center');
  FPGA_SETUP_BL1 : rtifpgainterfacelib/FPGA_SETUP_BL1  DSProperties=struct('RTI',struct('Version',uint32(15),'BlockType',struct('isSLSource',uint8(0),'isSLSink',uint8(0),'isHWSource',uint8(0),'isHWSink',uint8(0),'isSetup',uint8(1),'isInline',uint8(1),'isNonInline',uint8(0),'isInterrupt',uint8(0),'isChannelwise',uint8(0)),'IOBoardType','DSFPGA','UnitType','SETUP','Identifier','SETUP','DialogType','ML','BlockSet','FPGA','SlaveProcessor',''))  RTIBlockInterface=struct('InitLevel',3,'DialogFcn','rtifpgasetupgui','BlockDisplay',{{['FPGA Setup'],'auto'}},'IconTransparency','off','BlockName',struct('Token',{{'FPGA_SETUP_BL1'}}))  RTIBlockParameters="struct('BoardNo',{{1,'OFF',[1 16]}},'BoardType',{{[' '],'OFF',[]}},'MaxNumIOModuleSlots',{{5,'OFF',[]}},'FrameDir',{{'MATLAB\\RTIFPGA\\FRAMEWORKS\\DS1302_XC7K325T_FLEXIBLEIO','OFF',[]}},'IOFrameworks',{{struct('Fullname','','Filename',''),'OFF',[]}},'MdlIniDir',{{'C:\\marcos\\LSPyC_Varios\\MG_mono\\MGmono_rtiFPGA/INI/fpga_4B1619CAFD331D.ini','OFF',[]}},'PiggyBack',{{'fpga_framework_ini_DS1302_XC7K325T_FLEXIBLEIO.p','OFF',[]}},'PiggyBackAdd',{{[' '],'OFF',[]}},'FpgaAppID',{{0,'OFF',[0 65535]}},'FpgaBuildOpt',{{1,'OFF',[1 4]}},'FpgaAppName',{{'\"fpga\"','OFF',[]}},'FpgaAppSamRate',{{'1','OFF',[]}},'FpgaOptBldDir',{{[' '],'OFF',[]}},'OfflineSimPeriod',{{'1e-08','OFF',[]}},'TmpFrmID',{{-1,'OFF',[]}},'RestrictUsage',{{0,'OFF',[0 1]}},'Description',{{[' '],'OFF',[]}},'FPGATraceEnabled',{{0,'OFF',[]}},'MaxNumSubClocks',{{10,'OFF',[0 20]}},'SubClocks',{{struct('Subsystem',[' '],'Period','1','OfflineSimPeriod','1'),'OFF',[]}},'MaxNumTraceSubSystems',{{8,'OFF',[0 20]}},'TraceSubSystems',{{[' '],'OFF',[]}},'FPGATraceSubSystems',{{0,'OFF',[]}},'FPGATracedSPACE',{{0,'OFF',[]}},'FPGATraceDelays',{{0,'OFF',[]}},'FPGATraceOthers',{{0,'OFF',[]}},'AutomaticFpgaAppName',{{1,'OFF',[]}},'AutomaticFpgaBldDir',{{1,'OFF',[]}},'ParallelBuild',{{1,'OFF',[]}},'NewCfgDskPrj',{{[' '],'OFF',[]}},'RecentCfgDskPrj',{{[' '],'OFF',[]}},'FPGATraceBlocks',{{0,'OFF',[]}},'FPGATraceCompleteBuses',{{0,'OFF',[]}},'FPGACalibEnabled',{{0,'OFF',[]}},'MCSubSystems',{{[' '],'OFF',[]}},'FPGATAEnabled',{{0,'OFF',[]}},'MdlIniDirNew',{{'C:\\marcos\\LSPyC_Varios\\MG_mono\\MGmono_rtiFPGA/INI/fpga_4B1619CAFD331D.ini','OFF',[]}},'MGTFrameworks',{{struct('Fullname','','Filename',''),'OFF',[]}},'AutomaticBusAnalysis',{{1,'OFF',[]}})"  RTISFcnParameters=struct('BoardNo','double')  RTIBlockParaDefault=struct('BoardNo',1,'BoardType',[' '],'MaxNumIOModuleSlots',5,'FrameDir',[' '],'IOFrameworks',struct('Fullname','','Filename',''),'MdlIniDir',[' '],'PiggyBack',[' '],'PiggyBackAdd',[' '],'FpgaAppID',0,'FpgaBuildOpt',1,'FpgaAppName','---','FpgaAppSamRate','1','FpgaOptBldDir',[' '],'OfflineSimPeriod','1','TmpFrmID',-1,'RestrictUsage',0,'Description',[' '],'FPGATraceEnabled',0,'MaxNumSubClocks',10,'SubClocks',struct('Subsystem',[' '],'Period','1','OfflineSimPeriod','1'),'MaxNumTraceSubSystems',8,'TraceSubSystems',[' '],'FPGATraceSubSystems',0,'FPGATracedSPACE',0,'FPGATraceDelays',0,'FPGATraceOthers',0,'AutomaticFpgaAppName',1,'AutomaticFpgaBldDir',1,'ParallelBuild',1,'NewCfgDskPrj',[' '],'RecentCfgDskPrj',[' '],'FPGATraceBlocks',0,'FPGATraceCompleteBuses',0,'FPGACalibEnabled',0,'MCSubSystems',[' '],'FPGATAEnabled',0,'MdlIniDirNew',[' '],'MGTFrameworks',struct('Fullname',[' '],'Filename',[' ']),'AutomaticBusAnalysis',1)
  FPGA_XDATA_READ_BL1 : Subsystem  LoadFcn=try, rti_fpga_blk_loadfcn(gcbh); catch,errordlg({lasterr, '','Please check your RTI installation.'},['Error: ' upper(bdroot)], 'replace'); end  InitFcn=try, rti_fpga_blk_initfcn(gcbh); catch,errordlg({lasterr, '','Please check your RTI installation.'},['Error: ' upper(bdroot)], 'replace'); end  StartFcn=try, rti_fpga_blk_startfcn(gcbh); catch,errordlg({lasterr, '','Please check your RTI installation.'},['Error: ' upper(bdroot)], 'replace'); end  mask(RTI){DSProperties=struct('RTI',struct('Version',uint32(5),'BlockType',struct('isSLSource',uint8(1),'isSLSink',uint8(0),'isHWSource',uint8(0),'isHWSink',uint8(0),'isSetup',uint8(1),'isInline',uint8(1),'isNonInline',uint8(0),'isInterrupt',uint8(0),'isChannelwise',uint8(0)),'IOBoardType','DSFPGA','UnitType','','Identifier','PHSREAD','DialogType','ML','BlockSet','FPGA','SlaveProcessor','')), RTIBlockInterface=struct('OutputPortsActive',1,'OutputPortsWidth',int32(1),'OutputPortsDataType',{{'SS_DOUBLE'}},'OutputPortsName',{{['From XDATA']}},'InitLevel',3,'DialogFcn','rtifpgaphsreadgui','BlockDisplay',{{['XDATA Read'],'auto'}},'IconTransparency','on','BlockName',struct('Token',{{'FPGA_XDATA_Read_BL1'}})), RTIBlockParameters=struct('BoardNo',{{1,'OFF',[1 16]}},'Name',{{['Register In 1'],'OFF',[]}},'CustomName',{{['d_pv '],'OFF',[]}},'AccessTyp',{{'Register','OFF',[]}},'ChannelNo',{{'1','OFF',[]}},'FrmIni',{{'fpga_framework_ini_DS1302_XC7K325T_FLEXIBLEIO','OFF',[]}},'DynFcn',{{struct('GUIPar',struct('Name',{{['Binary point position (or fraction width)']},{'Format'},{['Register Group ID']},{['Enable simulation port']},{['Simulation ports sample time']},{['Used Flag']}},'GUIType',{{'edit'},{'popup','signed','unsigned','floating-point'},{'edit'},{'checkbox'},{'edit'},{'none'}},'Range',{{[0 1 2 3 4 5 6 7 8 9 10 11 12 13 14 15 16 17 18 19 20 21 22 23 24 25 26 27 28 29 30 31 32]},{'signed','unsigned','floating-point'},{[0 1 2 3 4 5 6 7 8 9 10 11 12 13 14 15 16 17 18 19 20 21 22 23 24 25 26 27 28 29 30 31 32 33 34 35 36 37 38 39 40 41 42 43 44 45 46 47 48 49 50 51 52 53 54 55 56 57 58 59 60 61 62 63]},{'0','1'},{''},{'0','1'}},'Init',{{'0'},{'signed'},{'0'},{'0'},{'-1','1'},{'1','0'}},'Group',{{''},{''},{''},{''},{''},{''}},'Generic',{{''},{''},{'xreg2fpga_group_000'},{''},{'REGISTER_IN_000_SIM_PORT_SAMPLE_TIME'},{'xreg2fpga_inst_000'}},'Application',{{''},{''},{''},{'ApplicationOut(1).Show'},{''},{''}},'Framework',{{'FrameworkIn(1).BinaryPoint'},{'FrameworkIn(1).Format'},{''},{''},{''},{''}},'Callback',{{'proc_bus_fpga_framework_ini_DS1302:fraction_width'},{'proc_bus_fpga_framework_ini_DS1302:fraction_width'},{''},{''},{''},{''}}),'Exl',{{''}},'HlpFile',{{'rtifpga','REGISTER_IN_DS1302'}},'Hlp',{{['Click below for further details on this I/O function.']}},'Gen',struct('name',{'','','xreg2fpga_group_000','','REGISTER_IN_000_SIM_PORT_SAMPLE_TIME','xreg2fpga_inst_000'},'value',{'','','1','','-1','1'},'unusedinit',{'','','','','1','0'},'tag',{'','','','','',''},'filename',{'','','','','',''}),'Frm',struct('FrameworkOut',struct('Name',{},'BitWidth',{},'BinaryPoint',{},'Format',{}),'FrameworkIn',struct('Name',{{'xreg_000_dout'},{'xreg_000_dout_wr'}},'BitWidth',{{'32'},{'1'}},'BinaryPoint',{{'0'},{'0'}},'Format',{{'unsigned'},{'unsigned'}},'DownSample',{[],{true}})),'App',struct('ApplicationOut',struct('Name',{{'Sim_Data'}},'Show',{{0}}),'ApplicationIn',struct('Name',{{'Data'},{['Data New']}},'Show',{{true},{true}})),'Con',{{'FrameworkIn(1)','ApplicationIn(1)','FrameworkIn(2)','ApplicationIn(2)'}},'OffCon',{{'data_o','FrameworkIn(1)','data_i','ApplicationOut(1)','data_new_o','FrameworkIn(2)'}},'OffModel',{{'phs_read_register'}}),'OFF',[]}},'FPGAFrameworkId',{{'8','OFF',[]}},'CorrBlock',{{struct('Data','','DataTag',''),'OFF',[]}},'BusSettings',{{[' '],'OFF',[]}}), RTISFcnParameters=struct('BoardNo','double'), RTIBlockParaDefault=struct('BoardNo',1,'Name',[' '],'CustomName',[' '],'AccessTyp',['<not selected>'],'ChannelNo',[' '],'FrmIni',[' '],'DynFcn',struct('GUIPar','','Hlp','','HlpFile','','Frm','','Gen','','Exl','','App','','Con',''),'FPGAFrameworkId',[' '],'CorrBlock',struct('Data','','DataTag',''),'BusSettings',[' '])}
      mask init:
      | % blkh = gcbh;
      | % [sfi, sfp, sfpt] = rti_fpga_blockinitial(blkh,'UPDATEPARAMETER');
      | % rti_fpga_blockinitial(blkh,'UPDATEBLOCKGUI');
      settings: CopyFcn=try, rti_fpga_blk_copyfcn(gcbh); catch,errordlg({lasterr, '','Please check your RTI installation.'},['Error: ' upper(bdroot)], 'replace'); end  DeleteFcn=try, rti_fpga_blk_deletefcn(gcbh); catch,errordlg({lasterr, '','Please check your RTI installation.'},['Error: ' upper(bdroot)], 'replace'); end  ModelCloseFcn=try, rti_fpga_blk_modelclosefcn(gcbh); catch,errordlg({lasterr, '','Please check your RTI installation.'},['Error: ' upper(bdroot)], 'replace'); end  PreSaveFcn=try, rti_fpga_blk_presavefcn(gcbh); catch,errordlg({lasterr, '','Please check your RTI installation.'},['Error: ' upper(bdroot)], 'replace'); end  NameChangeFcn=try, rti_fpga_blk_namechangefcn(gcbh); catch,errordlg({lasterr, '','Please check your RTI installation.'},['Error: ' upper(bdroot)], 'replace'); end  OpenFcn=try, rti_fpga_blk_openfcn(gcbh); catch,errordlg({lasterr, '','Please check your RTI installation.'},['Error: ' upper(bdroot)], 'replace'); end  CloseFcn=try, rti_fpga_blk_closefcn(gcbh); catch,errordlg({lasterr, '','Please check your RTI installation.'},['Error: ' upper(bdroot)], 'replace'); end  ParentCloseFcn=try, rti_fpga_blk_parentclosefcn(gcbh); catch,errordlg({lasterr, '','Please check your RTI installation.'},['Error: ' upper(bdroot)], 'replace'); end
      mask Help: eval( ['lasterror(''reset''); rtifpgaguilib(''RTIMaskHelp'', gcbh);', 'disp(lasterr);']);
      mask Display: text(0.5,0.65,'Register In 1','HorizontalAlignment','center');text(0.5,0.5,'d_pv ','HorizontalAlignment','center');text(0.5,0.35,'Group: 1','HorizontalAlignment','center');
  FPGA_XDATA_READ_BL2 : Subsystem  LoadFcn=try, rti_fpga_blk_loadfcn(gcbh); catch,errordlg({lasterr, '','Please check your RTI installation.'},['Error: ' upper(bdroot)], 'replace'); end  InitFcn=try, rti_fpga_blk_initfcn(gcbh); catch,errordlg({lasterr, '','Please check your RTI installation.'},['Error: ' upper(bdroot)], 'replace'); end  StartFcn=try, rti_fpga_blk_startfcn(gcbh); catch,errordlg({lasterr, '','Please check your RTI installation.'},['Error: ' upper(bdroot)], 'replace'); end  mask(RTI){DSProperties=struct('RTI',struct('Version',uint32(5),'BlockType',struct('isSLSource',uint8(1),'isSLSink',uint8(0),'isHWSource',uint8(0),'isHWSink',uint8(0),'isSetup',uint8(1),'isInline',uint8(1),'isNonInline',uint8(0),'isInterrupt',uint8(0),'isChannelwise',uint8(0)),'IOBoardType','DSFPGA','UnitType','','Identifier','PHSREAD','DialogType','ML','BlockSet','FPGA','SlaveProcessor','')), RTIBlockInterface=struct('OutputPortsActive',1,'OutputPortsWidth',int32(1),'OutputPortsDataType',{{'SS_DOUBLE'}},'OutputPortsName',{{['From XDATA']}},'InitLevel',3,'DialogFcn','rtifpgaphsreadgui','BlockDisplay',{{['XDATA Read'],'auto'}},'IconTransparency','on','BlockName',struct('Token',{{'FPGA_XDATA_Read_BL1'}})), RTIBlockParameters=struct('BoardNo',{{1,'OFF',[1 16]}},'Name',{{['Register In 2'],'OFF',[]}},'CustomName',{{'d_bat','OFF',[]}},'AccessTyp',{{'Register','OFF',[]}},'ChannelNo',{{'2','OFF',[]}},'FrmIni',{{'fpga_framework_ini_DS1302_XC7K325T_FLEXIBLEIO','OFF',[]}},'DynFcn',{{struct('GUIPar',struct('Name',{{['Binary point position (or fraction width)']},{'Format'},{['Register Group ID']},{['Enable simulation port']},{['Simulation ports sample time']},{['Used Flag']}},'GUIType',{{'edit'},{'popup','signed','unsigned','floating-point'},{'edit'},{'checkbox'},{'edit'},{'none'}},'Range',{{[0 1 2 3 4 5 6 7 8 9 10 11 12 13 14 15 16 17 18 19 20 21 22 23 24 25 26 27 28 29 30 31 32]},{'signed','unsigned','floating-point'},{[0 1 2 3 4 5 6 7 8 9 10 11 12 13 14 15 16 17 18 19 20 21 22 23 24 25 26 27 28 29 30 31 32 33 34 35 36 37 38 39 40 41 42 43 44 45 46 47 48 49 50 51 52 53 54 55 56 57 58 59 60 61 62 63]},{'0','1'},{''},{'0','1'}},'Init',{{'0'},{'signed'},{'0'},{'0'},{'-1','1'},{'1','0'}},'Group',{{''},{''},{''},{''},{''},{''}},'Generic',{{''},{''},{'xreg2fpga_group_001'},{''},{'REGISTER_IN_001_SIM_PORT_SAMPLE_TIME'},{'xreg2fpga_inst_001'}},'Application',{{''},{''},{''},{'ApplicationOut(1).Show'},{''},{''}},'Framework',{{'FrameworkIn(1).BinaryPoint'},{'FrameworkIn(1).Format'},{''},{''},{''},{''}},'Callback',{{'proc_bus_fpga_framework_ini_DS1302:fraction_width'},{'proc_bus_fpga_framework_ini_DS1302:fraction_width'},{''},{''},{''},{''}}),'Exl',{{''}},'HlpFile',{{'rtifpga','REGISTER_IN_DS1302'}},'Hlp',{{['Click below for further details on this I/O function.']}},'Gen',struct('name',{'','','xreg2fpga_group_001','','REGISTER_IN_001_SIM_PORT_SAMPLE_TIME','xreg2fpga_inst_001'},'value',{'','','1','','-1','1'},'unusedinit',{'','','','','1','0'},'tag',{'','','','','',''},'filename',{'','','','','',''}),'Frm',struct('FrameworkOut',struct('Name',{},'BitWidth',{},'BinaryPoint',{},'Format',{}),'FrameworkIn',struct('Name',{{'xreg_001_dout'},{'xreg_001_dout_wr'}},'BitWidth',{{'32'},{'1'}},'BinaryPoint',{{'0'},{'0'}},'Format',{{'unsigned'},{'unsigned'}},'DownSample',{[],{true}})),'App',struct('ApplicationOut',struct('Name',{{'Sim_Data'}},'Show',{{0}}),'ApplicationIn',struct('Name',{{'Data'},{['Data New']}},'Show',{{true},{true}})),'Con',{{'FrameworkIn(1)','ApplicationIn(1)','FrameworkIn(2)','ApplicationIn(2)'}},'OffCon',{{'data_o','FrameworkIn(1)','data_i','ApplicationOut(1)','data_new_o','FrameworkIn(2)'}},'OffModel',{{'phs_read_register'}}),'OFF',[]}},'FPGAFrameworkId',{{'8','OFF',[]}},'CorrBlock',{{struct('Data','','DataTag',''),'OFF',[]}},'BusSettings',{{[' '],'OFF',[]}}), RTISFcnParameters=struct('BoardNo','double'), RTIBlockParaDefault=struct('BoardNo',1,'Name',[' '],'CustomName',[' '],'AccessTyp',['<not selected>'],'ChannelNo',[' '],'FrmIni',[' '],'DynFcn',struct('GUIPar','','Hlp','','HlpFile','','Frm','','Gen','','Exl','','App','','Con',''),'FPGAFrameworkId',[' '],'CorrBlock',struct('Data','','DataTag',''),'BusSettings',[' '])}
      mask init:
      | % blkh = gcbh;
      | % [sfi, sfp, sfpt] = rti_fpga_blockinitial(blkh,'UPDATEPARAMETER');
      | % rti_fpga_blockinitial(blkh,'UPDATEBLOCKGUI');
      settings: CopyFcn=try, rti_fpga_blk_copyfcn(gcbh); catch,errordlg({lasterr, '','Please check your RTI installation.'},['Error: ' upper(bdroot)], 'replace'); end  DeleteFcn=try, rti_fpga_blk_deletefcn(gcbh); catch,errordlg({lasterr, '','Please check your RTI installation.'},['Error: ' upper(bdroot)], 'replace'); end  ModelCloseFcn=try, rti_fpga_blk_modelclosefcn(gcbh); catch,errordlg({lasterr, '','Please check your RTI installation.'},['Error: ' upper(bdroot)], 'replace'); end  PreSaveFcn=try, rti_fpga_blk_presavefcn(gcbh); catch,errordlg({lasterr, '','Please check your RTI installation.'},['Error: ' upper(bdroot)], 'replace'); end  NameChangeFcn=try, rti_fpga_blk_namechangefcn(gcbh); catch,errordlg({lasterr, '','Please check your RTI installation.'},['Error: ' upper(bdroot)], 'replace'); end  OpenFcn=try, rti_fpga_blk_openfcn(gcbh); catch,errordlg({lasterr, '','Please check your RTI installation.'},['Error: ' upper(bdroot)], 'replace'); end  CloseFcn=try, rti_fpga_blk_closefcn(gcbh); catch,errordlg({lasterr, '','Please check your RTI installation.'},['Error: ' upper(bdroot)], 'replace'); end  ParentCloseFcn=try, rti_fpga_blk_parentclosefcn(gcbh); catch,errordlg({lasterr, '','Please check your RTI installation.'},['Error: ' upper(bdroot)], 'replace'); end
      mask Help: eval( ['lasterror(''reset''); rtifpgaguilib(''RTIMaskHelp'', gcbh);', 'disp(lasterr);']);
      mask Display: text(0.5,0.65,'Register In 2','HorizontalAlignment','center');text(0.5,0.5,'d_bat','HorizontalAlignment','center');text(0.5,0.35,'Group: 1','HorizontalAlignment','center');
  FPGA_XDATA_READ_BL3 : Subsystem  LoadFcn=try, rti_fpga_blk_loadfcn(gcbh); catch,errordlg({lasterr, '','Please check your RTI installation.'},['Error: ' upper(bdroot)], 'replace'); end  InitFcn=try, rti_fpga_blk_initfcn(gcbh); catch,errordlg({lasterr, '','Please check your RTI installation.'},['Error: ' upper(bdroot)], 'replace'); end  StartFcn=try, rti_fpga_blk_startfcn(gcbh); catch,errordlg({lasterr, '','Please check your RTI installation.'},['Error: ' upper(bdroot)], 'replace'); end  mask(RTI){DSProperties=struct('RTI',struct('Version',uint32(5),'BlockType',struct('isSLSource',uint8(1),'isSLSink',uint8(0),'isHWSource',uint8(0),'isHWSink',uint8(0),'isSetup',uint8(1),'isInline',uint8(1),'isNonInline',uint8(0),'isInterrupt',uint8(0),'isChannelwise',uint8(0)),'IOBoardType','DSFPGA','UnitType','','Identifier','PHSREAD','DialogType','ML','BlockSet','FPGA','SlaveProcessor','')), RTIBlockInterface=struct('OutputPortsActive',1,'OutputPortsWidth',int32(1),'OutputPortsDataType',{{'SS_DOUBLE'}},'OutputPortsName',{{['From XDATA']}},'InitLevel',3,'DialogFcn','rtifpgaphsreadgui','BlockDisplay',{{['XDATA Read'],'auto'}},'IconTransparency','on','BlockName',struct('Token',{{'FPGA_XDATA_Read_BL1'}})), RTIBlockParameters=struct('BoardNo',{{1,'OFF',[1 16]}},'Name',{{['Register In 3'],'OFF',[]}},'CustomName',{{'d_vsi','OFF',[]}},'AccessTyp',{{'Register','OFF',[]}},'ChannelNo',{{'3','OFF',[]}},'FrmIni',{{'fpga_framework_ini_DS1302_XC7K325T_FLEXIBLEIO','OFF',[]}},'DynFcn',{{struct('GUIPar',struct('Name',{{['Binary point position (or fraction width)']},{'Format'},{['Register Group ID']},{['Enable simulation port']},{['Simulation ports sample time']},{['Used Flag']}},'GUIType',{{'edit'},{'popup','signed','unsigned','floating-point'},{'edit'},{'checkbox'},{'edit'},{'none'}},'Range',{{[0 1 2 3 4 5 6 7 8 9 10 11 12 13 14 15 16 17 18 19 20 21 22 23 24 25 26 27 28 29 30 31 32]},{'signed','unsigned','floating-point'},{[0 1 2 3 4 5 6 7 8 9 10 11 12 13 14 15 16 17 18 19 20 21 22 23 24 25 26 27 28 29 30 31 32 33 34 35 36 37 38 39 40 41 42 43 44 45 46 47 48 49 50 51 52 53 54 55 56 57 58 59 60 61 62 63]},{'0','1'},{''},{'0','1'}},'Init',{{'0'},{'signed'},{'0'},{'0'},{'-1','1'},{'1','0'}},'Group',{{''},{''},{''},{''},{''},{''}},'Generic',{{''},{''},{'xreg2fpga_group_002'},{''},{'REGISTER_IN_002_SIM_PORT_SAMPLE_TIME'},{'xreg2fpga_inst_002'}},'Application',{{''},{''},{''},{'ApplicationOut(1).Show'},{''},{''}},'Framework',{{'FrameworkIn(1).BinaryPoint'},{'FrameworkIn(1).Format'},{''},{''},{''},{''}},'Callback',{{'proc_bus_fpga_framework_ini_DS1302:fraction_width'},{'proc_bus_fpga_framework_ini_DS1302:fraction_width'},{''},{''},{''},{''}}),'Exl',{{''}},'HlpFile',{{'rtifpga','REGISTER_IN_DS1302'}},'Hlp',{{['Click below for further details on this I/O function.']}},'Gen',struct('name',{'','','xreg2fpga_group_002','','REGISTER_IN_002_SIM_PORT_SAMPLE_TIME','xreg2fpga_inst_002'},'value',{'','','1','','-1','1'},'unusedinit',{'','','','','1','0'},'tag',{'','','','','',''},'filename',{'','','','','',''}),'Frm',struct('FrameworkOut',struct('Name',{},'BitWidth',{},'BinaryPoint',{},'Format',{}),'FrameworkIn',struct('Name',{{'xreg_002_dout'},{'xreg_002_dout_wr'}},'BitWidth',{{'32'},{'1'}},'BinaryPoint',{{'0'},{'0'}},'Format',{{'unsigned'},{'unsigned'}},'DownSample',{[],{true}})),'App',struct('ApplicationOut',struct('Name',{{'Sim_Data'}},'Show',{{0}}),'ApplicationIn',struct('Name',{{'Data'},{['Data New']}},'Show',{{true},{true}})),'Con',{{'FrameworkIn(1)','ApplicationIn(1)','FrameworkIn(2)','ApplicationIn(2)'}},'OffCon',{{'data_o','FrameworkIn(1)','data_i','ApplicationOut(1)','data_new_o','FrameworkIn(2)'}},'OffModel',{{'phs_read_register'}}),'OFF',[]}},'FPGAFrameworkId',{{'8','OFF',[]}},'CorrBlock',{{struct('Data','','DataTag',''),'OFF',[]}},'BusSettings',{{[' '],'OFF',[]}}), RTISFcnParameters=struct('BoardNo','double'), RTIBlockParaDefault=struct('BoardNo',1,'Name',[' '],'CustomName',[' '],'AccessTyp',['<not selected>'],'ChannelNo',[' '],'FrmIni',[' '],'DynFcn',struct('GUIPar','','Hlp','','HlpFile','','Frm','','Gen','','Exl','','App','','Con',''),'FPGAFrameworkId',[' '],'CorrBlock',struct('Data','','DataTag',''),'BusSettings',[' '])}
      mask init:
      | % blkh = gcbh;
      | % [sfi, sfp, sfpt] = rti_fpga_blockinitial(blkh,'UPDATEPARAMETER');
      | % rti_fpga_blockinitial(blkh,'UPDATEBLOCKGUI');
      settings: CopyFcn=try, rti_fpga_blk_copyfcn(gcbh); catch,errordlg({lasterr, '','Please check your RTI installation.'},['Error: ' upper(bdroot)], 'replace'); end  DeleteFcn=try, rti_fpga_blk_deletefcn(gcbh); catch,errordlg({lasterr, '','Please check your RTI installation.'},['Error: ' upper(bdroot)], 'replace'); end  ModelCloseFcn=try, rti_fpga_blk_modelclosefcn(gcbh); catch,errordlg({lasterr, '','Please check your RTI installation.'},['Error: ' upper(bdroot)], 'replace'); end  PreSaveFcn=try, rti_fpga_blk_presavefcn(gcbh); catch,errordlg({lasterr, '','Please check your RTI installation.'},['Error: ' upper(bdroot)], 'replace'); end  NameChangeFcn=try, rti_fpga_blk_namechangefcn(gcbh); catch,errordlg({lasterr, '','Please check your RTI installation.'},['Error: ' upper(bdroot)], 'replace'); end  OpenFcn=try, rti_fpga_blk_openfcn(gcbh); catch,errordlg({lasterr, '','Please check your RTI installation.'},['Error: ' upper(bdroot)], 'replace'); end  CloseFcn=try, rti_fpga_blk_closefcn(gcbh); catch,errordlg({lasterr, '','Please check your RTI installation.'},['Error: ' upper(bdroot)], 'replace'); end  ParentCloseFcn=try, rti_fpga_blk_parentclosefcn(gcbh); catch,errordlg({lasterr, '','Please check your RTI installation.'},['Error: ' upper(bdroot)], 'replace'); end
      mask Help: eval( ['lasterror(''reset''); rtifpgaguilib(''RTIMaskHelp'', gcbh);', 'disp(lasterr);']);
      mask Display: text(0.5,0.65,'Register In 3','HorizontalAlignment','center');text(0.5,0.5,'d_vsi','HorizontalAlignment','center');text(0.5,0.35,'Group: 1','HorizontalAlignment','center');
  Terminator{,1..7} (8 alike) : Terminator
  wires:
  Black Box2/3 -> FPGA_INT_BL3/1(Int)
  FPGA_IO_WRITE_BL5/1(Data In) -> Terminator7/1
  FPGA_IO_WRITE_BL4/1(Data In) -> Terminator6/1
  Black Box2/2 -> FPGA_IO_WRITE_BL5/1(Data Out)
  Constant2/1 -> FPGA_IO_WRITE_BL4/2(Enable), FPGA_IO_WRITE_BL4/3(Direction), FPGA_IO_WRITE_BL5/2(Enable), FPGA_IO_WRITE_BL5/3(Direction)
  Black Box2/1 -> FPGA_IO_WRITE_BL4/1(Data Out)
  Black Box1/3 -> FPGA_INT_BL2/1(Int)
  FPGA_IO_WRITE_BL3/1(Data In) -> Terminator5/1
  Black Box1/2 -> FPGA_IO_WRITE_BL3/1(Data Out)
  FPGA_IO_WRITE_BL2/1(Data In) -> Terminator4/1
  Constant1/1 -> FPGA_IO_WRITE_BL2/3(Direction), FPGA_IO_WRITE_BL3/2(Enable), FPGA_IO_WRITE_BL3/3(Direction), FPGA_IO_WRITE_BL2/2(Enable)
  Black Box1/1 -> FPGA_IO_WRITE_BL2/1(Data Out)
  Black Box/2 -> FPGA_INT_BL1/1(Int)
  FPGA_IO_WRITE_BL1/1(Data In) -> Terminator3/1
  Constant/1 -> FPGA_IO_WRITE_BL1/2(Enable), FPGA_IO_WRITE_BL1/3(Direction)
  Black Box/1 -> FPGA_IO_WRITE_BL1/1(Data Out)
  FPGA_XDATA_READ_BL3/2(Data New) -> Terminator2/1
  FPGA_XDATA_READ_BL3/1(Data) -> Convert2/1
  FPGA_XDATA_READ_BL2/2(Data New) -> Terminator1/1
  FPGA_XDATA_READ_BL2/1(Data) -> Convert1/1
  FPGA_XDATA_READ_BL1/2(Data New) -> Terminator/1
  FPGA_XDATA_READ_BL1/1(Data) -> Convert/1
  Convert2/1 -> Black Box2/1
  Convert1/1 -> Black Box1/1
  Convert/1 -> Black Box/1
